simulink model "DYN_03x"  (R2021a)
(part 9 of 9)

C62 = 0.5*I6xx*de5*cos(e5)*sin(e4) - 0.5*I6xx*de4*cos(e4)*sin(e5) + 0.5*I6yy*de4*cos(e4)*sin(e5) - 0.5*I6yy*de5*cos(e5)*sin(e4) + I6zz*de4*cos(e4)*sin(e5) + I6zz*de5*cos(e5)*sin(e4) - 1.0*de2*m6*x6*y6*cos(e4)^2 + de2*m6*x6*y6*cos(e5)^2 - 1.0*de3*m6*x6*y6*cos(e4)^2 + de3*m6*x6*y6*cos(e5)^2 + 0.5*I6xx*de1*cos(e2)*cos(e3)*cos(e5) - 0.5*I6yy*de1*cos(e2)*cos(e3)*cos(e5) + I6xx*de2*cos(e4)*cos(e5)*sin(e4) + I6xx*de3*cos(e4)*cos(e5)*sin(e4) - 1.0*I6xx*de5*cos(e4)*cos(e6)*sin(e6) - 1.0*I6yy*de2*cos(e4)*cos(e5)*sin(e4) - 1.0*I6yy*de3*cos(e4)*cos(e5)*sin(e4) + I6yy*de5*cos(e4)*cos(e6)*sin(e6) - 0.5*I6xx*de1*cos(e5)*sin(e2)*sin(e3) + 0.5*I6yy*de1*cos(e5)*sin(e2)*sin(e3) + 1.5*de4*m6*x6^2*cos(e4)*sin(e5) + 0.5*de5*m6*x6^2*cos(e5)*sin(e4) + 0.5*de4*m6*y6^2*cos(e4)*sin(e5) + 1.5*de5*m6*y6^2*cos(e5)*sin(e4) - 1.0*I6xx*de2*cos(e4)^2*cos(e6)*sin(e6) + I6xx*de2*cos(e5)^2*cos(e6)*sin(e6) - 1.0*I6xx*de3*cos(e4)^2*cos(e6)*sin(e6) + I6xx*de4*cos(e4)*cos(e6)^2*sin(e5) + I6xx*de3*cos(e5)^2*cos(e6)*sin(e6) - 1.0*I6xx*de5*cos(e5)*cos(e6)^2*sin(e4) + I6yy*de2*cos(e4)^2*cos(e6)*sin(e6) - 1.0*I6yy*de2*cos(e5)^2*cos(e6)*sin(e6) + I6yy*de3*cos(e4)^2*cos(e6)*sin(e6) - 1.0*I6yy*de4*cos(e4)*cos(e6)^2*sin(e5) - 1.0*I6yy*de3*cos(e5)^2*cos(e6)*sin(e6) + I6yy*de5*cos(e5)*cos(e6)^2*sin(e4) - 1.0*de5*m6*x6*y6*cos(e4) + 2.0*de5*m6*x6*y6*cos(e4)*cos(e6)^2 + 0.5*I6xx*de1*cos(e2)*cos(e4)*sin(e3)*sin(e5) + 0.5*I6xx*de1*cos(e3)*cos(e4)*sin(e2)*sin(e5) - 0.5*I6yy*de1*cos(e2)*cos(e4)*sin(e3)*sin(e5) - 0.5*I6yy*de1*cos(e3)*cos(e4)*sin(e2)*sin(e5) - 0.5*de1*m6*x6^2*cos(e2)*cos(e3)*cos(e5) + 0.5*de1*m6*y6^2*cos(e2)*cos(e3)*cos(e5) - 1.0*de2*m6*x6^2*cos(e4)*cos(e5)*sin(e4) - 1.0*de3*m6*x6^2*cos(e4)*cos(e5)*sin(e4) + de5*m6*x6^2*cos(e4)*cos(e6)*sin(e6) - 1.0*de2*m6*x6*y6*cos(e4)^2*cos(e5)^2 + 2.0*de2*m6*x6*y6*cos(e4)^2*cos(e6)^2 - 1.0*de3*m6*x6*y6*cos(e4)^2*cos(e5)^2 - 2.0*de2*m6*x6*y6*cos(e5)^2*cos(e6)^2 + 2.0*de3*m6*x6*y6*cos(e4)^2*cos(e6)^2 - 2.0*de3*m6*x6*y6*cos(e5)^2*cos(e6)^2 + de2*m6*y6^2*cos(e4)*cos(e5)*sin(e4) + de3*m6*y6^2*cos(e4)*cos(e5)*sin(e4) - 1.0*de5*m6*y6^2*cos(e4)*cos(e6)*sin(e6) + 0.5*de1*m6*x6^2*cos(e5)*sin(e2)*sin(e3) - 0.5*de1*m6*y6^2*cos(e5)*sin(e2)*sin(e3) - 1.0*I6xx*de1*cos(e2)*cos(e3)*cos(e4)^2*cos(e5) - 1.0*I6xx*de1*cos(e2)*cos(e3)*cos(e5)*cos(e6)^2 + I6yy*de1*cos(e2)*cos(e3)*cos(e4)^2*cos(e5) + I6yy*de1*cos(e2)*cos(e3)*cos(e5)*cos(e6)^2 - 0.5*a3*de5*m6*y6*cos(e5)*cos(e6) + 0.5*d4*de4*m6*x6*cos(e4)*cos(e6) - 2.0*I6xx*de2*cos(e4)*cos(e5)*cos(e6)^2*sin(e4) - 2.0*I6xx*de3*cos(e4)*cos(e5)*cos(e6)^2*sin(e4) + 2.0*I6yy*de2*cos(e4)*cos(e5)*cos(e6)^2*sin(e4) + 2.0*I6yy*de3*cos(e4)*cos(e5)*cos(e6)^2*sin(e4) + a3*de2*m6*x6*cos(e6)*sin(e4) + a3*de3*m6*x6*cos(e6)*sin(e4) - 0.5*a3*de5*m6*x6*cos(e5)*sin(e6) - 0.5*a3*de6*m6*x6*cos(e6)*sin(e5) + I6xx*de1*cos(e4)^2*cos(e5)*sin(e2)*sin(e3) + I6xx*de1*cos(e5)*cos(e6)^2*sin(e2)*sin(e3) - 1.0*I6yy*de1*cos(e4)^2*cos(e5)*sin(e2)*sin(e3) - 1.0*I6yy*de1*cos(e5)*cos(e6)^2*sin(e2)*sin(e3) + d4*de2*m6*y6*cos(e6)*sin(e5) + d4*de3*m6*y6*cos(e6)*sin(e5) - 0.5*d4*de4*m6*y6*cos(e4)*sin(e6) - 0.5*d4*de6*m6*y6*cos(e6)*sin(e4) + 0.5*de6*m6*x6*z6*cos(e4)*cos(e6) - 1.0*a3*de2*m6*y6*sin(e4)*sin(e6) - 1.0*a3*de3*m6*y6*sin(e4)*sin(e6) + 0.5*a3*de6*m6*y6*sin(e5)*sin(e6) + d4*de2*m6*x6*sin(e5)*sin(e6) + d4*de3*m6*x6*sin(e5)*sin(e6) - 0.5*d4*de6*m6*x6*sin(e4)*sin(e6) - 1.5*de4*m6*y6*z6*cos(e6)*sin(e4) - 0.5*de6*m6*y6*z6*cos(e4)*sin(e6) + de2*m6*x6^2*cos(e4)^2*cos(e6)*sin(e6) - 1.0*de2*m6*x6^2*cos(e5)^2*cos(e6)*sin(e6) + de3*m6*x6^2*cos(e4)^2*cos(e6)*sin(e6) - 1.0*de4*m6*x6^2*cos(e4)*cos(e6)^2*sin(e5) - 1.0*de3*m6*x6^2*cos(e5)^2*cos(e6)*sin(e6) + de5*m6*x6^2*cos(e5)*cos(e6)^2*sin(e4) - 1.0*de2*m6*y6^2*cos(e4)^2*cos(e6)*sin(e6) + de2*m6*y6^2*cos(e5)^2*cos(e6)*sin(e6) - 1.0*de3*m6*y6^2*cos(e4)^2*cos(e6)*sin(e6) + de4*m6*y6^2*cos(e4)*cos(e6)^2*sin(e5) + de3*m6*y6^2*cos(e5)^2*cos(e6)*sin(e6) - 1.0*de5*m6*y6^2*cos(e5)*cos(e6)^2*sin(e4) - 1.5*de4*m6*x6*z6*sin(e4)*sin(e6) - 1.0*I6xx*de2*cos(e4)^2*cos(e5)^2*cos(e6)*sin(e6) - 1.0*I6xx*de3*cos(e4)^2*cos(e5)^2*cos(e6)*sin(e6) + I6yy*de2*cos(e4)^2*cos(e5)^2*cos(e6)*sin(e6) + I6yy*de3*cos(e4)^2*cos(e5)^2*cos(e6)*sin(e6) - 1.0*I6xx*de4*cos(e5)*cos(e6)*sin(e4)*sin(e5)*sin(e6) + I6yy*de4*cos(e5)*cos(e6)*sin(e4)*sin(e5)*sin(e6) - 0.5*de1*m6*x6^2*cos(e2)*cos(e4)*sin(e3)*sin(e5) - 0.5*de1*m6*x6^2*cos(e3)*cos(e4)*sin(e2)*sin(e5) + 0.5*de1*m6*y6^2*cos(e2)*cos(e4)*sin(e3)*sin(e5) + 0.5*de1*m6*y6^2*cos(e3)*cos(e4)*sin(e2)*sin(e5) - 0.5*a2*de1*m6*x6*cos(e2)*cos(e4)*cos(e6) + a3*de2*m6*y6*cos(e4)*cos(e5)*cos(e6) - 0.5*a2*de5*m6*y6*cos(e3)*cos(e5)*cos(e6) + a3*de3*m6*y6*cos(e4)*cos(e5)*cos(e6) + 0.5*d4*de6*m6*x6*cos(e4)*cos(e5)*cos(e6) + a2*de2*m6*x6*cos(e3)*cos(e6)*sin(e4) - 0.5*a2*de3*m6*x6*cos(e3)*cos(e6)*sin(e4) - 0.5*a2*de4*m6*x6*cos(e4)*cos(e6)*sin(e3) + a3*de2*m6*x6*cos(e4)*cos(e5)*sin(e6) - 0.5*a2*de5*m6*x6*cos(e3)*cos(e5)*sin(e6) + a3*de3*m6*x6*cos(e4)*cos(e5)*sin(e6) - 0.5*a2*de6*m6*x6*cos(e3)*cos(e6)*sin(e5) + 0.5*a2*de1*m6*y6*cos(e2)*cos(e4)*sin(e6) - 1.0*I6xx*de1*cos(e2)*cos(e4)*cos(e6)^2*sin(e3)*sin(e5) - 1.0*I6xx*de1*cos(e3)*cos(e4)*cos(e6)^2*sin(e2)*sin(e5) + I6yy*de1*cos(e2)*cos(e4)*cos(e6)^2*sin(e3)*sin(e5) + I6yy*de1*cos(e3)*cos(e4)*cos(e6)^2*sin(e2)*sin(e5) - 0.5*d4*de4*m6*y6*cos(e5)*cos(e6)*sin(e4) - 0.5*d4*de5*m6*y6*cos(e4)*cos(e6)*sin(e5) - 0.5*d4*de6*m6*y6*cos(e4)*cos(e5)*sin(e6) + 0.5*de4*m6*x6*z6*cos(e4)*cos(e5)*cos(e6) - 1.0*a2*de2*m6*y6*cos(e3)*sin(e4)*sin(e6) - 1.0*a2*de2*m6*y6*cos(e6)*sin(e3)*sin(e5) + 0.5*a2*de3*m6*y6*cos(e3)*sin(e4)*sin(e6) + 0.5*a2*de3*m6*y6*cos(e6)*sin(e3)*sin(e5) + 0.5*a2*de4*m6*y6*cos(e4)*sin(e3)*sin(e6) + 0.5*a2*de6*m6*y6*cos(e6)*sin(e3)*sin(e4) + 0.5*a2*de6*m6*y6*cos(e3)*sin(e5)*sin(e6) - 0.5*d4*de4*m6*x6*cos(e5)*sin(e4)*sin(e6) - 0.5*d4*de5*m6*x6*cos(e4)*sin(e5)*sin(e6) + de1*m6*x6^2*cos(e2)*cos(e3)*cos(e4)^2*cos(e5) + de1*m6*x6^2*cos(e2)*cos(e3)*cos(e5)*cos(e6)^2 - 1.0*de1*m6*y6^2*cos(e2)*cos(e3)*cos(e4)^2*cos(e5) - 1.0*de1*m6*y6^2*cos(e2)*cos(e3)*cos(e5)*cos(e6)^2 + de2*m6*y6*z6*cos(e5)*cos(e6)*sin(e5) + de3*m6*y6*z6*cos(e5)*cos(e6)*sin(e5) - 0.5*de4*m6*y6*z6*cos(e4)*cos(e5)*sin(e6) - 0.5*de6*m6*y6*z6*cos(e5)*cos(e6)*sin(e4) - 1.0*a2*de2*m6*x6*sin(e3)*sin(e5)*sin(e6) + 0.5*a2*de3*m6*x6*sin(e3)*sin(e5)*sin(e6) + 0.5*a2*de6*m6*x6*sin(e3)*sin(e4)*sin(e6) + 2.0*de2*m6*x6^2*cos(e4)*cos(e5)*cos(e6)^2*sin(e4) + 2.0*de3*m6*x6^2*cos(e4)*cos(e5)*cos(e6)^2*sin(e4) + 2.0*de2*m6*x6*y6*cos(e4)^2*cos(e5)^2*cos(e6)^2 + 2.0*de3*m6*x6*y6*cos(e4)^2*cos(e5)^2*cos(e6)^2 - 2.0*de2*m6*y6^2*cos(e4)*cos(e5)*cos(e6)^2*sin(e4) - 2.0*de3*m6*y6^2*cos(e4)*cos(e5)*cos(e6)^2*sin(e4) - 1.0*de4*m6*x6*y6*cos(e5)*sin(e4)*sin(e5) + de2*m6*x6*z6*cos(e5)*sin(e5)*sin(e6) + de3*m6*x6*z6*cos(e5)*sin(e5)*sin(e6) - 1.5*de5*m6*x6*z6*cos(e6)*sin(e4)*sin(e5) - 0.5*de6*m6*x6*z6*cos(e5)*sin(e4)*sin(e6) - 1.0*de1*m6*x6^2*cos(e4)^2*cos(e5)*sin(e2)*sin(e3) - 1.0*de1*m6*x6^2*cos(e5)*cos(e6)^2*sin(e2)*sin(e3) + de1*m6*y6^2*cos(e4)^2*cos(e5)*sin(e2)*sin(e3) + de1*m6*y6^2*cos(e5)*cos(e6)^2*sin(e2)*sin(e3) + 1.5*de5*m6*y6*z6*sin(e4)*sin(e5)*sin(e6) + 2.0*I6xx*de1*cos(e2)*cos(e3)*cos(e4)^2*cos(e5)*cos(e6)^2 - 2.0*I6yy*de1*cos(e2)*cos(e3)*cos(e4)^2*cos(e5)*cos(e6)^2 - 2.0*I6xx*de1*cos(e4)^2*cos(e5)*cos(e6)^2*sin(e2)*sin(e3) + 2.0*I6yy*de1*cos(e4)^2*cos(e5)*cos(e6)^2*sin(e2)*sin(e3) + de4*m6*y6*z6*cos(e5)^2*cos(e6)*sin(e4) + de2*m6*x6^2*cos(e4)^2*cos(e5)^2*cos(e6)*sin(e6) + de3*m6*x6^2*cos(e4)^2*cos(e5)^2*cos(e6)*sin(e6) - 1.0*de2*m6*y6^2*cos(e4)^2*cos(e5)^2*cos(e6)*sin(e6) - 1.0*de3*m6*y6^2*cos(e4)^2*cos(e5)^2*cos(e6)*sin(e6) + de4*m6*x6*z6*cos(e5)^2*sin(e4)*sin(e6) + de4*m6*x6^2*cos(e5)*cos(e6)*sin(e4)*sin(e5)*sin(e6) - 1.0*de4*m6*y6^2*cos(e5)*cos(e6)*sin(e4)*sin(e5)*sin(e6) - 0.5*a3*de1*m6*x6*cos(e2)*cos(e3)*cos(e4)*cos(e6) + a2*de2*m6*y6*cos(e3)*cos(e4)*cos(e5)*cos(e6) - 0.5*a2*de3*m6*y6*cos(e3)*cos(e4)*cos(e5)*cos(e6) + a2*de2*m6*x6*cos(e3)*cos(e4)*cos(e5)*sin(e6) - 0.5*a2*de3*m6*x6*cos(e3)*cos(e4)*cos(e5)*sin(e6) - 0.5*a2*de6*m6*x6*cos(e4)*cos(e5)*cos(e6)*sin(e3) + 0.5*a3*de1*m6*y6*cos(e2)*cos(e3)*cos(e4)*sin(e6) + 0.5*a2*de1*m6*y6*cos(e2)*cos(e5)*cos(e6)*sin(e4) + 0.5*d4*de1*m6*x6*cos(e2)*cos(e4)*cos(e6)*sin(e3) + 0.5*d4*de1*m6*x6*cos(e3)*cos(e4)*cos(e6)*sin(e2) + 0.5*a3*de1*m6*x6*cos(e4)*cos(e6)*sin(e2)*sin(e3) + 0.5*a2*de1*m6*x6*cos(e2)*cos(e5)*sin(e4)*sin(e6) + 0.5*a2*de4*m6*y6*cos(e5)*cos(e6)*sin(e3)*sin(e4) + 0.5*a2*de5*m6*y6*cos(e4)*cos(e6)*sin(e3)*sin(e5) + 0.5*a2*de6*m6*y6*cos(e4)*cos(e5)*sin(e3)*sin(e6) - 0.5*d4*de1*m6*y6*cos(e2)*cos(e4)*sin(e3)*sin(e6) - 0.5*d4*de1*m6*y6*cos(e3)*cos(e4)*sin(e2)*sin(e6) - 1.0*de1*m6*x6*y6*cos(e2)*cos(e3)*cos(e4)*sin(e4) - 0.5*de1*m6*x6*z6*cos(e2)*cos(e3)*cos(e6)*sin(e5) + 0.5*a2*de4*m6*x6*cos(e5)*sin(e3)*sin(e4)*sin(e6) + 0.5*a2*de5*m6*x6*cos(e4)*sin(e3)*sin(e5)*sin(e6) - 0.5*a3*de1*m6*y6*cos(e4)*sin(e2)*sin(e3)*sin(e6) + 2.0*de4*m6*x6*y6*cos(e4)*cos(e6)*sin(e5)*sin(e6) - 2.0*de5*m6*x6*y6*cos(e5)*cos(e6)*sin(e4)*sin(e6) - 1.0*de2*m6*x6*z6*cos(e4)*cos(e6)*sin(e4)*sin(e5) - 1.0*de3*m6*x6*z6*cos(e4)*cos(e6)*sin(e4)*sin(e5) + 0.5*de1*m6*y6*z6*cos(e2)*cos(e6)*sin(e3)*sin(e4) + 0.5*de1*m6*y6*z6*cos(e3)*cos(e6)*sin(e2)*sin(e4) + 0.5*de1*m6*y6*z6*cos(e2)*cos(e3)*sin(e5)*sin(e6) + de1*m6*x6^2*cos(e2)*cos(e4)*cos(e6)^2*sin(e3)*sin(e5) + de1*m6*x6^2*cos(e3)*cos(e4)*cos(e6)^2*sin(e2)*sin(e5) - 1.0*de1*m6*y6^2*cos(e2)*cos(e4)*cos(e6)^2*sin(e3)*sin(e5) - 1.0*de1*m6*y6^2*cos(e3)*cos(e4)*cos(e6)^2*sin(e2)*sin(e5) + de1*m6*x6*y6*cos(e4)*sin(e2)*sin(e3)*sin(e4) + 0.5*de1*m6*x6*z6*cos(e2)*sin(e3)*sin(e4)*sin(e6) + 0.5*de1*m6*x6*z6*cos(e3)*sin(e2)*sin(e4)*sin(e6) + 0.5*de1*m6*x6*z6*cos(e6)*sin(e2)*sin(e3)*sin(e5) + de2*m6*y6*z6*cos(e4)*sin(e4)*sin(e5)*sin(e6) + de3*m6*y6*z6*cos(e4)*sin(e4)*sin(e5)*sin(e6) - 0.5*de1*m6*y6*z6*sin(e2)*sin(e3)*sin(e5)*sin(e6) - 2.0*de1*m6*x6^2*cos(e2)*cos(e3)*cos(e4)^2*cos(e5)*cos(e6)^2 + 2.0*de1*m6*y6^2*cos(e2)*cos(e3)*cos(e4)^2*cos(e5)*cos(e6)^2 - 1.0*de2*m6*y6*z6*cos(e4)^2*cos(e5)*cos(e6)*sin(e5) - 1.0*de3*m6*y6*z6*cos(e4)^2*cos(e5)*cos(e6)*sin(e5) + 2.0*de4*m6*x6*y6*cos(e5)*cos(e6)^2*sin(e4)*sin(e5) - 1.0*de2*m6*x6*z6*cos(e4)^2*cos(e5)*sin(e5)*sin(e6) - 1.0*de3*m6*x6*z6*cos(e4)^2*cos(e5)*sin(e5)*sin(e6) + 2.0*de1*m6*x6^2*cos(e4)^2*cos(e5)*cos(e6)^2*sin(e2)*sin(e3) - 2.0*de1*m6*y6^2*cos(e4)^2*cos(e5)*cos(e6)^2*sin(e2)*sin(e3) - 1.0*I6xx*de1*cos(e2)*cos(e3)*cos(e4)*cos(e6)*sin(e4)*sin(e6) + I6yy*de1*cos(e2)*cos(e3)*cos(e4)*cos(e6)*sin(e4)*sin(e6) + I6xx*de1*cos(e4)*cos(e6)*sin(e2)*sin(e3)*sin(e4)*sin(e6) - 1.0*I6yy*de1*cos(e4)*cos(e6)*sin(e2)*sin(e3)*sin(e4)*sin(e6) + 0.5*a3*de1*m6*y6*cos(e2)*cos(e3)*cos(e5)*cos(e6)*sin(e4) - 1.0*I6xx*de1*cos(e2)*cos(e3)*cos(e4)*cos(e5)^2*cos(e6)*sin(e4)*sin(e6) + I6yy*de1*cos(e2)*cos(e3)*cos(e4)*cos(e5)^2*cos(e6)*sin(e4)*sin(e6) + 0.5*a3*de1*m6*x6*cos(e2)*cos(e3)*cos(e5)*sin(e4)*sin(e6) - 0.5*d4*de1*m6*y6*cos(e2)*cos(e5)*cos(e6)*sin(e3)*sin(e4) - 0.5*d4*de1*m6*y6*cos(e3)*cos(e5)*cos(e6)*sin(e2)*sin(e4) - 2.0*de1*m6*x6*y6*cos(e2)*cos(e3)*cos(e5)*cos(e6)*sin(e6) + 0.5*de1*m6*x6*z6*cos(e2)*cos(e4)*cos(e5)*cos(e6)*sin(e3) + 0.5*de1*m6*x6*z6*cos(e3)*cos(e4)*cos(e5)*cos(e6)*sin(e2) - 0.5*a3*de1*m6*y6*cos(e5)*cos(e6)*sin(e2)*sin(e3)*sin(e4) - 0.5*d4*de1*m6*x6*cos(e2)*cos(e5)*sin(e3)*sin(e4)*sin(e6) - 0.5*d4*de1*m6*x6*cos(e3)*cos(e5)*sin(e2)*sin(e4)*sin(e6) + I6xx*de1*cos(e4)*cos(e5)^2*cos(e6)*sin(e2)*sin(e3)*sin(e4)*sin(e6) - 1.0*I6yy*de1*cos(e4)*cos(e5)^2*cos(e6)*sin(e2)*sin(e3)*sin(e4)*sin(e6) - 4.0*de2*m6*x6*y6*cos(e4)*cos(e5)*cos(e6)*sin(e4)*sin(e6) - 4.0*de3*m6*x6*y6*cos(e4)*cos(e5)*cos(e6)*sin(e4)*sin(e6) - 0.5*de1*m6*y6*z6*cos(e2)*cos(e4)*cos(e5)*sin(e3)*sin(e6) - 0.5*de1*m6*y6*z6*cos(e3)*cos(e4)*cos(e5)*sin(e2)*sin(e6) - 0.5*a3*de1*m6*x6*cos(e5)*sin(e2)*sin(e3)*sin(e4)*sin(e6) + de1*m6*x6*y6*cos(e2)*cos(e5)*sin(e3)*sin(e4)*sin(e5) + de1*m6*x6*y6*cos(e3)*cos(e5)*sin(e2)*sin(e4)*sin(e5) + 2.0*de1*m6*x6*y6*cos(e5)*cos(e6)*sin(e2)*sin(e3)*sin(e6) - 1.0*de1*m6*x6*y6*cos(e2)*cos(e3)*cos(e4)*cos(e5)^2*sin(e4) + 2.0*de1*m6*x6*y6*cos(e2)*cos(e3)*cos(e4)*cos(e6)^2*sin(e4) + de1*m6*x6*z6*cos(e2)*cos(e3)*cos(e4)^2*cos(e6)*sin(e5) - 1.0*de1*m6*y6*z6*cos(e2)*cos(e3)*cos(e4)^2*sin(e5)*sin(e6) - 1.0*de1*m6*y6*z6*cos(e2)*cos(e5)^2*cos(e6)*sin(e3)*sin(e4) - 1.0*de1*m6*y6*z6*cos(e3)*cos(e5)^2*cos(e6)*sin(e2)*sin(e4) + de1*m6*x6*y6*cos(e4)*cos(e5)^2*sin(e2)*sin(e3)*sin(e4) - 2.0*de1*m6*x6*y6*cos(e4)*cos(e6)^2*sin(e2)*sin(e3)*sin(e4) - 1.0*de1*m6*x6*z6*cos(e2)*cos(e5)^2*sin(e3)*sin(e4)*sin(e6) - 1.0*de1*m6*x6*z6*cos(e3)*cos(e5)^2*sin(e2)*sin(e4)*sin(e6) - 1.0*de1*m6*x6*z6*cos(e4)^2*cos(e6)*sin(e2)*sin(e3)*sin(e5) + de1*m6*y6*z6*cos(e4)^2*sin(e2)*sin(e3)*sin(e5)*sin(e6) + I6xx*de1*cos(e2)*cos(e5)*cos(e6)*sin(e3)*sin(e4)*sin(e5)*sin(e6) + I6xx*de1*cos(e3)*cos(e5)*cos(e6)*sin(e2)*sin(e4)*sin(e5)*sin(e6) - 1.0*I6yy*de1*cos(e2)*cos(e5)*cos(e6)*sin(e3)*sin(e4)*sin(e5)*sin(e6) - 1.0*I6yy*de1*cos(e3)*cos(e5)*cos(e6)*sin(e2)*sin(e4)*sin(e5)*sin(e6) + de1*m6*x6^2*cos(e2)*cos(e3)*cos(e4)*cos(e6)*sin(e4)*sin(e6) - 1.0*de1*m6*y6^2*cos(e2)*cos(e3)*cos(e4)*cos(e6)*sin(e4)*sin(e6) - 1.0*de1*m6*x6^2*cos(e4)*cos(e6)*sin(e2)*sin(e3)*sin(e4)*sin(e6) + de1*m6*y6^2*cos(e4)*cos(e6)*sin(e2)*sin(e3)*sin(e4)*sin(e6) + de1*m6*x6^2*cos(e2)*cos(e3)*cos(e4)*cos(e5)^2*cos(e6)*sin(e4)*sin(e6) - 1.0*de1*m6*y6^2*cos(e2)*cos(e3)*cos(e4)*cos(e5)^2*cos(e6)*sin(e4)*sin(e6) - 2.0*de1*m6*x6*y6*cos(e2)*cos(e4)*cos(e6)*sin(e3)*sin(e5)*sin(e6) - 2.0*de1*m6*x6*y6*cos(e3)*cos(e4)*cos(e6)*sin(e2)*sin(e5)*sin(e6) - 1.0*de1*m6*x6^2*cos(e4)*cos(e5)^2*cos(e6)*sin(e2)*sin(e3)*sin(e4)*sin(e6) + de1*m6*y6^2*cos(e4)*cos(e5)^2*cos(e6)*sin(e2)*sin(e3)*sin(e4)*sin(e6) + 4.0*de1*m6*x6*y6*cos(e2)*cos(e3)*cos(e4)^2*cos(e5)*cos(e6)*sin(e6) - 2.0*de1*m6*x6*y6*cos(e2)*cos(e5)*cos(e6)^2*sin(e3)*sin(e4)*sin(e5) - 2.0*de1*m6*x6*y6*cos(e3)*cos(e5)*cos(e6)^2*sin(e2)*sin(e4)*sin(e5) - 4.0*de1*m6*x6*y6*cos(e4)^2*cos(e5)*cos(e6)*sin(e2)*sin(e3)*sin(e6) + 2.0*de1*m6*x6*y6*cos(e2)*cos(e3)*cos(e4)*cos(e5)^2*cos(e6)^2*sin(e4) - 1.0*de1*m6*x6^2*cos(e2)*cos(e5)*cos(e6)*sin(e3)*sin(e4)*sin(e5)*sin(e6) - 1.0*de1*m6*x6^2*cos(e3)*cos(e5)*cos(e6)*sin(e2)*sin(e4)*sin(e5)*sin(e6) - 2.0*de1*m6*x6*y6*cos(e4)*cos(e5)^2*cos(e6)^2*sin(e2)*sin(e3)*sin(e4) + de1*m6*y6^2*cos(e2)*cos(e5)*cos(e6)*sin(e3)*sin(e4)*sin(e5)*sin(e6) + de1*m6*y6^2*cos(e3)*cos(e5)*cos(e6)*sin(e2)*sin(e4)*sin(e5)*sin(e6) - 1.0*de1*m6*y6*z6*cos(e2)*cos(e3)*cos(e4)*cos(e5)*cos(e6)*sin(e4)*sin(e5) - 1.0*de1*m6*x6*z6*cos(e2)*cos(e3)*cos(e4)*cos(e5)*sin(e4)*sin(e5)*sin(e6) + de1*m6*y6*z6*cos(e4)*cos(e5)*cos(e6)*sin(e2)*sin(e3)*sin(e4)*sin(e5) + de1*m6*x6*z6*cos(e4)*cos(e5)*sin(e2)*sin(e3)*sin(e4)*sin(e5)*sin(e6);
C63 = 0.5*I6xx*de5*cos(e5)*sin(e4) - 0.5*I6xx*de4*cos(e4)*sin(e5) + 0.5*I6yy*de4*cos(e4)*sin(e5) - 0.5*I6yy*de5*cos(e5)*sin(e4) + I6zz*de4*cos(e4)*sin(e5) + I6zz*de5*cos(e5)*sin(e4) - 1.0*de2*m6*x6*y6*cos(e4)^2 + de2*m6*x6*y6*cos(e5)^2 - 1.0*de3*m6*x6*y6*cos(e4)^2 + de3*m6*x6*y6*cos(e5)^2 + 0.5*I6xx*de1*cos(e2)*cos(e3)*cos(e5) - 0.5*I6yy*de1*cos(e2)*cos(e3)*cos(e5) + I6xx*de2*cos(e4)*cos(e5)*sin(e4) + I6xx*de3*cos(e4)*cos(e5)*sin(e4) - 1.0*I6xx*de5*cos(e4)*cos(e6)*sin(e6) - 1.0*I6yy*de2*cos(e4)*cos(e5)*sin(e4) - 1.0*I6yy*de3*cos(e4)*cos(e5)*sin(e4) + I6yy*de5*cos(e4)*cos(e6)*sin(e6) - 0.5*I6xx*de1*cos(e5)*sin(e2)*sin(e3) + 0.5*I6yy*de1*cos(e5)*sin(e2)*sin(e3) + 1.5*de4*m6*x6^2*cos(e4)*sin(e5) + 0.5*de5*m6*x6^2*cos(e5)*sin(e4) + 0.5*de4*m6*y6^2*cos(e4)*sin(e5) + 1.5*de5*m6*y6^2*cos(e5)*sin(e4) - 1.0*I6xx*de2*cos(e4)^2*cos(e6)*sin(e6) + I6xx*de2*cos(e5)^2*cos(e6)*sin(e6) - 1.0*I6xx*de3*cos(e4)^2*cos(e6)*sin(e6) + I6xx*de4*cos(e4)*cos(e6)^2*sin(e5) + I6xx*de3*cos(e5)^2*cos(e6)*sin(e6) - 1.0*I6xx*de5*cos(e5)*cos(e6)^2*sin(e4) + I6yy*de2*cos(e4)^2*cos(e6)*sin(e6) - 1.0*I6yy*de2*cos(e5)^2*cos(e6)*sin(e6) + I6yy*de3*cos(e4)^2*cos(e6)*sin(e6) - 1.0*I6yy*de4*cos(e4)*cos(e6)^2*sin(e5) - 1.0*I6yy*de3*cos(e5)^2*cos(e6)*sin(e6) + I6yy*de5*cos(e5)*cos(e6)^2*sin(e4) - 1.0*de5*m6*x6*y6*cos(e4) + 2.0*de5*m6*x6*y6*cos(e4)*cos(e6)^2 + 0.5*I6xx*de1*cos(e2)*cos(e4)*sin(e3)*sin(e5) + 0.5*I6xx*de1*cos(e3)*cos(e4)*sin(e2)*sin(e5) - 0.5*I6yy*de1*cos(e2)*cos(e4)*sin(e3)*sin(e5) - 0.5*I6yy*de1*cos(e3)*cos(e4)*sin(e2)*sin(e5) - 0.5*de1*m6*x6^2*cos(e2)*cos(e3)*cos(e5) + 0.5*de1*m6*y6^2*cos(e2)*cos(e3)*cos(e5) - 1.0*de2*m6*x6^2*cos(e4)*cos(e5)*sin(e4) - 1.0*de3*m6*x6^2*cos(e4)*cos(e5)*sin(e4) + de5*m6*x6^2*cos(e4)*cos(e6)*sin(e6) - 1.0*de2*m6*x6*y6*cos(e4)^2*cos(e5)^2 + 2.0*de2*m6*x6*y6*cos(e4)^2*cos(e6)^2 - 1.0*de3*m6*x6*y6*cos(e4)^2*cos(e5)^2 - 2.0*de2*m6*x6*y6*cos(e5)^2*cos(e6)^2 + 2.0*de3*m6*x6*y6*cos(e4)^2*cos(e6)^2 - 2.0*de3*m6*x6*y6*cos(e5)^2*cos(e6)^2 + de2*m6*y6^2*cos(e4)*cos(e5)*sin(e4) + de3*m6*y6^2*cos(e4)*cos(e5)*sin(e4) - 1.0*de5*m6*y6^2*cos(e4)*cos(e6)*sin(e6) + 0.5*de1*m6*x6^2*cos(e5)*sin(e2)*sin(e3) - 0.5*de1*m6*y6^2*cos(e5)*sin(e2)*sin(e3) - 1.0*I6xx*de1*cos(e2)*cos(e3)*cos(e4)^2*cos(e5) - 1.0*I6xx*de1*cos(e2)*cos(e3)*cos(e5)*cos(e6)^2 + I6yy*de1*cos(e2)*cos(e3)*cos(e4)^2*cos(e5) + I6yy*de1*cos(e2)*cos(e3)*cos(e5)*cos(e6)^2 - 0.5*a3*de5*m6*y6*cos(e5)*cos(e6) + 0.5*d4*de4*m6*x6*cos(e4)*cos(e6) - 2.0*I6xx*de2*cos(e4)*cos(e5)*cos(e6)^2*sin(e4) - 2.0*I6xx*de3*cos(e4)*cos(e5)*cos(e6)^2*sin(e4) + 2.0*I6yy*de2*cos(e4)*cos(e5)*cos(e6)^2*sin(e4) + 2.0*I6yy*de3*cos(e4)*cos(e5)*cos(e6)^2*sin(e4) + a3*de2*m6*x6*cos(e6)*sin(e4) + a3*de3*m6*x6*cos(e6)*sin(e4) - 0.5*a3*de5*m6*x6*cos(e5)*sin(e6) - 0.5*a3*de6*m6*x6*cos(e6)*sin(e5) + I6xx*de1*cos(e4)^2*cos(e5)*sin(e2)*sin(e3) + I6xx*de1*cos(e5)*cos(e6)^2*sin(e2)*sin(e3) - 1.0*I6yy*de1*cos(e4)^2*cos(e5)*sin(e2)*sin(e3) - 1.0*I6yy*de1*cos(e5)*cos(e6)^2*sin(e2)*sin(e3) + d4*de2*m6*y6*cos(e6)*sin(e5) + d4*de3*m6*y6*cos(e6)*sin(e5) - 0.5*d4*de4*m6*y6*cos(e4)*sin(e6) - 0.5*d4*de6*m6*y6*cos(e6)*sin(e4) + 0.5*de6*m6*x6*z6*cos(e4)*cos(e6) - 1.0*a3*de2*m6*y6*sin(e4)*sin(e6) - 1.0*a3*de3*m6*y6*sin(e4)*sin(e6) + 0.5*a3*de6*m6*y6*sin(e5)*sin(e6) + d4*de2*m6*x6*sin(e5)*sin(e6) + d4*de3*m6*x6*sin(e5)*sin(e6) - 0.5*d4*de6*m6*x6*sin(e4)*sin(e6) - 1.5*de4*m6*y6*z6*cos(e6)*sin(e4) - 0.5*de6*m6*y6*z6*cos(e4)*sin(e6) + de2*m6*x6^2*cos(e4)^2*cos(e6)*sin(e6) - 1.0*de2*m6*x6^2*cos(e5)^2*cos(e6)*sin(e6) + de3*m6*x6^2*cos(e4)^2*cos(e6)*sin(e6) - 1.0*de4*m6*x6^2*cos(e4)*cos(e6)^2*sin(e5) - 1.0*de3*m6*x6^2*cos(e5)^2*cos(e6)*sin(e6) + de5*m6*x6^2*cos(e5)*cos(e6)^2*sin(e4) - 1.0*de2*m6*y6^2*cos(e4)^2*cos(e6)*sin(e6) + de2*m6*y6^2*cos(e5)^2*cos(e6)*sin(e6) - 1.0*de3*m6*y6^2*cos(e4)^2*cos(e6)*sin(e6) + de4*m6*y6^2*cos(e4)*cos(e6)^2*sin(e5) + de3*m6*y6^2*cos(e5)^2*cos(e6)*sin(e6) - 1.0*de5*m6*y6^2*cos(e5)*cos(e6)^2*sin(e4) - 1.5*de4*m6*x6*z6*sin(e4)*sin(e6) - 1.0*I6xx*de2*cos(e4)^2*cos(e5)^2*cos(e6)*sin(e6) - 1.0*I6xx*de3*cos(e4)^2*cos(e5)^2*cos(e6)*sin(e6) + I6yy*de2*cos(e4)^2*cos(e5)^2*cos(e6)*sin(e6) + I6yy*de3*cos(e4)^2*cos(e5)^2*cos(e6)*sin(e6) - 1.0*I6xx*de4*cos(e5)*cos(e6)*sin(e4)*sin(e5)*sin(e6) + I6yy*de4*cos(e5)*cos(e6)*sin(e4)*sin(e5)*sin(e6) - 0.5*de1*m6*x6^2*cos(e2)*cos(e4)*sin(e3)*sin(e5) - 0.5*de1*m6*x6^2*cos(e3)*cos(e4)*sin(e2)*sin(e5) + 0.5*de1*m6*y6^2*cos(e2)*cos(e4)*sin(e3)*sin(e5) + 0.5*de1*m6*y6^2*cos(e3)*cos(e4)*sin(e2)*sin(e5) + a3*de2*m6*y6*cos(e4)*cos(e5)*cos(e6) + a3*de3*m6*y6*cos(e4)*cos(e5)*cos(e6) + 0.5*d4*de6*m6*x6*cos(e4)*cos(e5)*cos(e6) + 0.5*a2*de2*m6*x6*cos(e3)*cos(e6)*sin(e4) + a3*de2*m6*x6*cos(e4)*cos(e5)*sin(e6) + a3*de3*m6*x6*cos(e4)*cos(e5)*sin(e6) - 1.0*I6xx*de1*cos(e2)*cos(e4)*cos(e6)^2*sin(e3)*sin(e5) - 1.0*I6xx*de1*cos(e3)*cos(e4)*cos(e6)^2*sin(e2)*sin(e5) + I6yy*de1*cos(e2)*cos(e4)*cos(e6)^2*sin(e3)*sin(e5) + I6yy*de1*cos(e3)*cos(e4)*cos(e6)^2*sin(e2)*sin(e5) - 0.5*d4*de4*m6*y6*cos(e5)*cos(e6)*sin(e4) - 0.5*d4*de5*m6*y6*cos(e4)*cos(e6)*sin(e5) - 0.5*d4*de6*m6*y6*cos(e4)*cos(e5)*sin(e6) + 0.5*de4*m6*x6*z6*cos(e4)*cos(e5)*cos(e6) - 0.5*a2*de2*m6*y6*cos(e3)*sin(e4)*sin(e6) - 0.5*a2*de2*m6*y6*cos(e6)*sin(e3)*sin(e5) - 0.5*d4*de4*m6*x6*cos(e5)*sin(e4)*sin(e6) - 0.5*d4*de5*m6*x6*cos(e4)*sin(e5)*sin(e6) + de1*m6*x6^2*cos(e2)*cos(e3)*cos(e4)^2*cos(e5) + de1*m6*x6^2*cos(e2)*cos(e3)*cos(e5)*cos(e6)^2 - 1.0*de1*m6*y6^2*cos(e2)*cos(e3)*cos(e4)^2*cos(e5) - 1.0*de1*m6*y6^2*cos(e2)*cos(e3)*cos(e5)*cos(e6)^2 + de2*m6*y6*z6*cos(e5)*cos(e6)*sin(e5) + de3*m6*y6*z6*cos(e5)*cos(e6)*sin(e5) - 0.5*de4*m6*y6*z6*cos(e4)*cos(e5)*sin(e6) - 0.5*de6*m6*y6*z6*cos(e5)*cos(e6)*sin(e4) - 0.5*a2*de2*m6*x6*sin(e3)*sin(e5)*sin(e6) + 2.0*de2*m6*x6^2*cos(e4)*cos(e5)*cos(e6)^2*sin(e4) + 2.0*de3*m6*x6^2*cos(e4)*cos(e5)*cos(e6)^2*sin(e4) + 2.0*de2*m6*x6*y6*cos(e4)^2*cos(e5)^2*cos(e6)^2 + 2.0*de3*m6*x6*y6*cos(e4)^2*cos(e5)^2*cos(e6)^2 - 2.0*de2*m6*y6^2*cos(e4)*cos(e5)*cos(e6)^2*sin(e4) - 2.0*de3*m6*y6^2*cos(e4)*cos(e5)*cos(e6)^2*sin(e4) - 1.0*de4*m6*x6*y6*cos(e5)*sin(e4)*sin(e5) + de2*m6*x6*z6*cos(e5)*sin(e5)*sin(e6) + de3*m6*x6*z6*cos(e5)*sin(e5)*sin(e6) - 1.5*de5*m6*x6*z6*cos(e6)*sin(e4)*sin(e5) - 0.5*de6*m6*x6*z6*cos(e5)*sin(e4)*sin(e6) - 1.0*de1*m6*x6^2*cos(e4)^2*cos(e5)*sin(e2)*sin(e3) - 1.0*de1*m6*x6^2*cos(e5)*cos(e6)^2*sin(e2)*sin(e3) + de1*m6*y6^2*cos(e4)^2*cos(e5)*sin(e2)*sin(e3) + de1*m6*y6^2*cos(e5)*cos(e6)^2*sin(e2)*sin(e3) + 1.5*de5*m6*y6*z6*sin(e4)*sin(e5)*sin(e6) + 2.0*I6xx*de1*cos(e2)*cos(e3)*cos(e4)^2*cos(e5)*cos(e6)^2 - 2.0*I6yy*de1*cos(e2)*cos(e3)*cos(e4)^2*cos(e5)*cos(e6)^2 - 2.0*I6xx*de1*cos(e4)^2*cos(e5)*cos(e6)^2*sin(e2)*sin(e3) + 2.0*I6yy*de1*cos(e4)^2*cos(e5)*cos(e6)^2*sin(e2)*sin(e3) + de4*m6*y6*z6*cos(e5)^2*cos(e6)*sin(e4) + de2*m6*x6^2*cos(e4)^2*cos(e5)^2*cos(e6)*sin(e6) + de3*m6*x6^2*cos(e4)^2*cos(e5)^2*cos(e6)*sin(e6) - 1.0*de2*m6*y6^2*cos(e4)^2*cos(e5)^2*cos(e6)*sin(e6) - 1.0*de3*m6*y6^2*cos(e4)^2*cos(e5)^2*cos(e6)*sin(e6) + de4*m6*x6*z6*cos(e5)^2*sin(e4)*sin(e6) + de4*m6*x6^2*cos(e5)*cos(e6)*sin(e4)*sin(e5)*sin(e6) - 1.0*de4*m6*y6^2*cos(e5)*cos(e6)*sin(e4)*sin(e5)*sin(e6) - 0.5*a3*de1*m6*x6*cos(e2)*cos(e3)*cos(e4)*cos(e6) + 0.5*a2*de2*m6*y6*cos(e3)*cos(e4)*cos(e5)*cos(e6) + 0.5*a2*de2*m6*x6*cos(e3)*cos(e4)*cos(e5)*sin(e6) + 0.5*a3*de1*m6*y6*cos(e2)*cos(e3)*cos(e4)*sin(e6) + 0.5*d4*de1*m6*x6*cos(e2)*cos(e4)*cos(e6)*sin(e3) + 0.5*d4*de1*m6*x6*cos(e3)*cos(e4)*cos(e6)*sin(e2) + 0.5*a3*de1*m6*x6*cos(e4)*cos(e6)*sin(e2)*sin(e3) - 0.5*d4*de1*m6*y6*cos(e2)*cos(e4)*sin(e3)*sin(e6) - 0.5*d4*de1*m6*y6*cos(e3)*cos(e4)*sin(e2)*sin(e6) - 1.0*de1*m6*x6*y6*cos(e2)*cos(e3)*cos(e4)*sin(e4) - 0.5*de1*m6*x6*z6*cos(e2)*cos(e3)*cos(e6)*sin(e5) - 0.5*a3*de1*m6*y6*cos(e4)*sin(e2)*sin(e3)*sin(e6) + 2.0*de4*m6*x6*y6*cos(e4)*cos(e6)*sin(e5)*sin(e6) - 2.0*de5*m6*x6*y6*cos(e5)*cos(e6)*sin(e4)*sin(e6) - 1.0*de2*m6*x6*z6*cos(e4)*cos(e6)*sin(e4)*sin(e5) - 1.0*de3*m6*x6*z6*cos(e4)*cos(e6)*sin(e4)*sin(e5) + 0.5*de1*m6*y6*z6*cos(e2)*cos(e6)*sin(e3)*sin(e4) + 0.5*de1*m6*y6*z6*cos(e3)*cos(e6)*sin(e2)*sin(e4) + 0.5*de1*m6*y6*z6*cos(e2)*cos(e3)*sin(e5)*sin(e6) + de1*m6*x6^2*cos(e2)*cos(e4)*cos(e6)^2*sin(e3)*sin(e5) + de1*m6*x6^2*cos(e3)*cos(e4)*cos(e6)^2*sin(e2)*sin(e5) - 1.0*de1*m6*y6^2*cos(e2)*cos(e4)*cos(e6)^2*sin(e3)*sin(e5) - 1.0*de1*m6*y6^2*cos(e3)*cos(e4)*cos(e6)^2*sin(e2)*sin(e5) + de1*m6*x6*y6*cos(e4)*sin(e2)*sin(e3)*sin(e4) + 0.5*de1*m6*x6*z6*cos(e2)*sin(e3)*sin(e4)*sin(e6) + 0.5*de1*m6*x6*z6*cos(e3)*sin(e2)*sin(e4)*sin(e6) + 0.5*de1*m6*x6*z6*cos(e6)*sin(e2)*sin(e3)*sin(e5) + de2*m6*y6*z6*cos(e4)*sin(e4)*sin(e5)*sin(e6) + de3*m6*y6*z6*cos(e4)*sin(e4)*sin(e5)*sin(e6) - 0.5*de1*m6*y6*z6*sin(e2)*sin(e3)*sin(e5)*sin(e6) - 2.0*de1*m6*x6^2*cos(e2)*cos(e3)*cos(e4)^2*cos(e5)*cos(e6)^2 + 2.0*de1*m6*y6^2*cos(e2)*cos(e3)*cos(e4)^2*cos(e5)*cos(e6)^2 - 1.0*de2*m6*y6*z6*cos(e4)^2*cos(e5)*cos(e6)*sin(e5) - 1.0*de3*m6*y6*z6*cos(e4)^2*cos(e5)*cos(e6)*sin(e5) + 2.0*de4*m6*x6*y6*cos(e5)*cos(e6)^2*sin(e4)*sin(e5) - 1.0*de2*m6*x6*z6*cos(e4)^2*cos(e5)*sin(e5)*sin(e6) - 1.0*de3*m6*x6*z6*cos(e4)^2*cos(e5)*sin(e5)*sin(e6) + 2.0*de1*m6*x6^2*cos(e4)^2*cos(e5)*cos(e6)^2*sin(e2)*sin(e3) - 2.0*de1*m6*y6^2*cos(e4)^2*cos(e5)*cos(e6)^2*sin(e2)*sin(e3) - 1.0*I6xx*de1*cos(e2)*cos(e3)*cos(e4)*cos(e6)*sin(e4)*sin(e6) + I6yy*de1*cos(e2)*cos(e3)*cos(e4)*cos(e6)*sin(e4)*sin(e6) + I6xx*de1*cos(e4)*cos(e6)*sin(e2)*sin(e3)*sin(e4)*sin(e6) - 1.0*I6yy*de1*cos(e4)*cos(e6)*sin(e2)*sin(e3)*sin(e4)*sin(e6) + 0.5*a3*de1*m6*y6*cos(e2)*cos(e3)*cos(e5)*cos(e6)*sin(e4) - 1.0*I6xx*de1*cos(e2)*cos(e3)*cos(e4)*cos(e5)^2*cos(e6)*sin(e4)*sin(e6) + I6yy*de1*cos(e2)*cos(e3)*cos(e4)*cos(e5)^2*cos(e6)*sin(e4)*sin(e6) + 0.5*a3*de1*m6*x6*cos(e2)*cos(e3)*cos(e5)*sin(e4)*sin(e6) - 0.5*d4*de1*m6*y6*cos(e2)*cos(e5)*cos(e6)*sin(e3)*sin(e4) - 0.5*d4*de1*m6*y6*cos(e3)*cos(e5)*cos(e6)*sin(e2)*sin(e4) - 2.0*de1*m6*x6*y6*cos(e2)*cos(e3)*cos(e5)*cos(e6)*sin(e6) + 0.5*de1*m6*x6*z6*cos(e2)*cos(e4)*cos(e5)*cos(e6)*sin(e3) + 0.5*de1*m6*x6*z6*cos(e3)*cos(e4)*cos(e5)*cos(e6)*sin(e2) - 0.5*a3*de1*m6*y6*cos(e5)*cos(e6)*sin(e2)*sin(e3)*sin(e4) - 0.5*d4*de1*m6*x6*cos(e2)*cos(e5)*sin(e3)*sin(e4)*sin(e6) - 0.5*d4*de1*m6*x6*cos(e3)*cos(e5)*sin(e2)*sin(e4)*sin(e6) + I6xx*de1*cos(e4)*cos(e5)^2*cos(e6)*sin(e2)*sin(e3)*sin(e4)*sin(e6) - 1.0*I6yy*de1*cos(e4)*cos(e5)^2*cos(e6)*sin(e2)*sin(e3)*sin(e4)*sin(e6) - 4.0*de2*m6*x6*y6*cos(e4)*cos(e5)*cos(e6)*sin(e4)*sin(e6) - 4.0*de3*m6*x6*y6*cos(e4)*cos(e5)*cos(e6)*sin(e4)*sin(e6) - 0.5*de1*m6*y6*z6*cos(e2)*cos(e4)*cos(e5)*sin(e3)*sin(e6) - 0.5*de1*m6*y6*z6*cos(e3)*cos(e4)*cos(e5)*sin(e2)*sin(e6) - 0.5*a3*de1*m6*x6*cos(e5)*sin(e2)*sin(e3)*sin(e4)*sin(e6) + de1*m6*x6*y6*cos(e2)*cos(e5)*sin(e3)*sin(e4)*sin(e5) + de1*m6*x6*y6*cos(e3)*cos(e5)*sin(e2)*sin(e4)*sin(e5) + 2.0*de1*m6*x6*y6*cos(e5)*cos(e6)*sin(e2)*sin(e3)*sin(e6) - 1.0*de1*m6*x6*y6*cos(e2)*cos(e3)*cos(e4)*cos(e5)^2*sin(e4) + 2.0*de1*m6*x6*y6*cos(e2)*cos(e3)*cos(e4)*cos(e6)^2*sin(e4) + de1*m6*x6*z6*cos(e2)*cos(e3)*cos(e4)^2*cos(e6)*sin(e5) - 1.0*de1*m6*y6*z6*cos(e2)*cos(e3)*cos(e4)^2*sin(e5)*sin(e6) - 1.0*de1*m6*y6*z6*cos(e2)*cos(e5)^2*cos(e6)*sin(e3)*sin(e4) - 1.0*de1*m6*y6*z6*cos(e3)*cos(e5)^2*cos(e6)*sin(e2)*sin(e4) + de1*m6*x6*y6*cos(e4)*cos(e5)^2*sin(e2)*sin(e3)*sin(e4) - 2.0*de1*m6*x6*y6*cos(e4)*cos(e6)^2*sin(e2)*sin(e3)*sin(e4) - 1.0*de1*m6*x6*z6*cos(e2)*cos(e5)^2*sin(e3)*sin(e4)*sin(e6) - 1.0*de1*m6*x6*z6*cos(e3)*cos(e5)^2*sin(e2)*sin(e4)*sin(e6) - 1.0*de1*m6*x6*z6*cos(e4)^2*cos(e6)*sin(e2)*sin(e3)*sin(e5) + de1*m6*y6*z6*cos(e4)^2*sin(e2)*sin(e3)*sin(e5)*sin(e6) + I6xx*de1*cos(e2)*cos(e5)*cos(e6)*sin(e3)*sin(e4)*sin(e5)*sin(e6) + I6xx*de1*cos(e3)*cos(e5)*cos(e6)*sin(e2)*sin(e4)*sin(e5)*sin(e6) - 1.0*I6yy*de1*cos(e2)*cos(e5)*cos(e6)*sin(e3)*sin(e4)*sin(e5)*sin(e6) - 1.0*I6yy*de1*cos(e3)*cos(e5)*cos(e6)*sin(e2)*sin(e4)*sin(e5)*sin(e6) + de1*m6*x6^2*cos(e2)*cos(e3)*cos(e4)*cos(e6)*sin(e4)*sin(e6) - 1.0*de1*m6*y6^2*cos(e2)*cos(e3)*cos(e4)*cos(e6)*sin(e4)*sin(e6) - 1.0*de1*m6*x6^2*cos(e4)*cos(e6)*sin(e2)*sin(e3)*sin(e4)*sin(e6) + de1*m6*y6^2*cos(e4)*cos(e6)*sin(e2)*sin(e3)*sin(e4)*sin(e6) + de1*m6*x6^2*cos(e2)*cos(e3)*cos(e4)*cos(e5)^2*cos(e6)*sin(e4)*sin(e6) - 1.0*de1*m6*y6^2*cos(e2)*cos(e3)*cos(e4)*cos(e5)^2*cos(e6)*sin(e4)*sin(e6) - 2.0*de1*m6*x6*y6*cos(e2)*cos(e4)*cos(e6)*sin(e3)*sin(e5)*sin(e6) - 2.0*de1*m6*x6*y6*cos(e3)*cos(e4)*cos(e6)*sin(e2)*sin(e5)*sin(e6) - 1.0*de1*m6*x6^2*cos(e4)*cos(e5)^2*cos(e6)*sin(e2)*sin(e3)*sin(e4)*sin(e6) + de1*m6*y6^2*cos(e4)*cos(e5)^2*cos(e6)*sin(e2)*sin(e3)*sin(e4)*sin(e6) + 4.0*de1*m6*x6*y6*cos(e2)*cos(e3)*cos(e4)^2*cos(e5)*cos(e6)*sin(e6) - 2.0*de1*m6*x6*y6*cos(e2)*cos(e5)*cos(e6)^2*sin(e3)*sin(e4)*sin(e5) - 2.0*de1*m6*x6*y6*cos(e3)*cos(e5)*cos(e6)^2*sin(e2)*sin(e4)*sin(e5) - 4.0*de1*m6*x6*y6*cos(e4)^2*cos(e5)*cos(e6)*sin(e2)*sin(e3)*sin(e6) + 2.0*de1*m6*x6*y6*cos(e2)*cos(e3)*cos(e4)*cos(e5)^2*cos(e6)^2*sin(e4) - 1.0*de1*m6*x6^2*cos(e2)*cos(e5)*cos(e6)*sin(e3)*sin(e4)*sin(e5)*sin(e6) - 1.0*de1*m6*x6^2*cos(e3)*cos(e5)*cos(e6)*sin(e2)*sin(e4)*sin(e5)*sin(e6) - 2.0*de1*m6*x6*y6*cos(e4)*cos(e5)^2*cos(e6)^2*sin(e2)*sin(e3)*sin(e4) + de1*m6*y6^2*cos(e2)*cos(e5)*cos(e6)*sin(e3)*sin(e4)*sin(e5)*sin(e6) + de1*m6*y6^2*cos(e3)*cos(e5)*cos(e6)*sin(e2)*sin(e4)*sin(e5)*sin(e6) - 1.0*de1*m6*y6*z6*cos(e2)*cos(e3)*cos(e4)*cos(e5)*cos(e6)*sin(e4)*sin(e5) - 1.0*de1*m6*x6*z6*cos(e2)*cos(e3)*cos(e4)*cos(e5)*sin(e4)*sin(e5)*sin(e6) + de1*m6*y6*z6*cos(e4)*cos(e5)*cos(e6)*sin(e2)*sin(e3)*sin(e4)*sin(e5) + de1*m6*x6*z6*cos(e4)*cos(e5)*sin(e2)*sin(e3)*sin(e4)*sin(e5)*sin(e6);
C64 = 0.25*I6xx*de4*sin(2.0*e6) - 0.25*I6yy*de4*sin(2.0*e6) - 0.5*I6xx*de5*sin(e5) + 0.5*I6yy*de5*sin(e5) - 1.0*I6zz*de5*sin(e5) + I6xx*de5*cos(e6)^2*sin(e5) - 1.0*I6yy*de5*cos(e6)^2*sin(e5) - 0.25*de4*m6*x6^2*sin(2.0*e6) + 0.25*de4*m6*y6^2*sin(2.0*e6) - 0.5*I6xx*de2*cos(e4)*sin(e5) - 0.5*I6xx*de3*cos(e4)*sin(e5) + 0.5*I6yy*de2*cos(e4)*sin(e5) + 0.5*I6yy*de3*cos(e4)*sin(e5) - 0.5*de5*m6*x6^2*sin(e5) - 1.5*de5*m6*y6^2*sin(e5) - 1.0*de5*m6*x6^2*cos(e6)^2*sin(e5) + de5*m6*y6^2*cos(e6)^2*sin(e5) - 0.5*I6xx*de4*cos(2.0*e5)*cos(e6)*sin(e6) + 0.5*I6yy*de4*cos(2.0*e5)*cos(e6)*sin(e6) - 0.5*de4*m6*x6*y6*cos(2.0*e5) - 0.5*de4*m6*x6*y6*cos(2.0*e6) + 0.5*de2*m6*x6^2*cos(e4)*sin(e5) + 0.5*de3*m6*x6^2*cos(e4)*sin(e5) - 0.5*de2*m6*y6^2*cos(e4)*sin(e5) - 0.5*de3*m6*y6^2*cos(e4)*sin(e5) + I6xx*de2*cos(e4)*cos(e6)^2*sin(e5) + I6xx*de3*cos(e4)*cos(e6)^2*sin(e5) - 1.0*I6yy*de2*cos(e4)*cos(e6)^2*sin(e5) - 1.0*I6yy*de3*cos(e4)*cos(e6)^2*sin(e5) + 0.5*de4*m6*x6^2*cos(2.0*e5)*cos(e6)*sin(e6) - 0.5*de4*m6*y6^2*cos(2.0*e5)*cos(e6)*sin(e6) - 0.5*I6xx*de1*cos(e2)*cos(e3)*sin(e4)*sin(e5) - 1.0*I6xx*de1*cos(e2)*cos(e6)*sin(e3)*sin(e6) - 1.0*I6xx*de1*cos(e3)*cos(e6)*sin(e2)*sin(e6) + 0.5*I6yy*de1*cos(e2)*cos(e3)*sin(e4)*sin(e5) + I6yy*de1*cos(e2)*cos(e6)*sin(e3)*sin(e6) + I6yy*de1*cos(e3)*cos(e6)*sin(e2)*sin(e6) - 0.5*de4*m6*y6*z6*sin(2.0*e5)*cos(e6) + 0.5*I6xx*de1*sin(e2)*sin(e3)*sin(e4)*sin(e5) - 0.5*I6yy*de1*sin(e2)*sin(e3)*sin(e4)*sin(e5) - 0.5*de4*m6*x6*z6*sin(2.0*e5)*sin(e6) - 0.5*d4*de2*m6*x6*cos(e4)*cos(e6) - 0.5*d4*de3*m6*x6*cos(e4)*cos(e6) - 0.5*a1*de1*m6*x6*cos(e6)*sin(e4) + 0.5*d4*de2*m6*y6*cos(e4)*sin(e6) + 0.5*d4*de3*m6*y6*cos(e4)*sin(e6) + de4*m6*x6*y6*cos(2.0*e5)*cos(e6)^2 - 1.5*de5*m6*x6*z6*cos(e5)*cos(e6) + 0.5*a1*de1*m6*y6*sin(e4)*sin(e6) - 1.0*de1*m6*x6*y6*cos(e2)*sin(e3) - 1.0*de1*m6*x6*y6*cos(e3)*sin(e2) - 0.5*de2*m6*y6*z6*cos(e6)*sin(e4) - 0.5*de3*m6*y6*z6*cos(e6)*sin(e4) + 1.5*de5*m6*y6*z6*cos(e5)*sin(e6) + 0.5*de6*m6*y6*z6*cos(e6)*sin(e5) - 1.0*de2*m6*x6^2*cos(e4)*cos(e6)^2*sin(e5) - 1.0*de3*m6*x6^2*cos(e4)*cos(e6)^2*sin(e5) + de2*m6*y6^2*cos(e4)*cos(e6)^2*sin(e5) + de3*m6*y6^2*cos(e4)*cos(e6)^2*sin(e5) - 0.5*de2*m6*x6*z6*sin(e4)*sin(e6) - 0.5*de3*m6*x6*z6*sin(e4)*sin(e6) + 0.5*de6*m6*x6*z6*sin(e5)*sin(e6) - 1.0*I6xx*de2*cos(e5)*cos(e6)*sin(e4)*sin(e5)*sin(e6) - 1.0*I6xx*de3*cos(e5)*cos(e6)*sin(e4)*sin(e5)*sin(e6) + I6yy*de2*cos(e5)*cos(e6)*sin(e4)*sin(e5)*sin(e6) + I6yy*de3*cos(e5)*cos(e6)*sin(e4)*sin(e5)*sin(e6) + 0.5*de1*m6*x6^2*cos(e2)*cos(e3)*sin(e4)*sin(e5) + de1*m6*x6^2*cos(e2)*cos(e6)*sin(e3)*sin(e6) + de1*m6*x6^2*cos(e3)*cos(e6)*sin(e2)*sin(e6) - 0.5*de1*m6*y6^2*cos(e2)*cos(e3)*sin(e4)*sin(e5) - 1.0*de1*m6*y6^2*cos(e2)*cos(e6)*sin(e3)*sin(e6) - 1.0*de1*m6*y6^2*cos(e3)*cos(e6)*sin(e2)*sin(e6) - 0.5*a1*de1*m6*y6*cos(e4)*cos(e5)*cos(e6) - 0.5*de1*m6*x6^2*sin(e2)*sin(e3)*sin(e4)*sin(e5) + 0.5*de1*m6*y6^2*sin(e2)*sin(e3)*sin(e4)*sin(e5) - 0.5*a1*de1*m6*x6*cos(e4)*cos(e5)*sin(e6) + 0.5*a2*de2*m6*x6*cos(e4)*cos(e6)*sin(e3) + I6xx*de1*cos(e2)*cos(e3)*cos(e6)^2*sin(e4)*sin(e5) + I6xx*de1*cos(e2)*cos(e5)^2*cos(e6)*sin(e3)*sin(e6) + I6xx*de1*cos(e3)*cos(e5)^2*cos(e6)*sin(e2)*sin(e6) - 1.0*I6yy*de1*cos(e2)*cos(e3)*cos(e6)^2*sin(e4)*sin(e5) - 1.0*I6yy*de1*cos(e2)*cos(e5)^2*cos(e6)*sin(e3)*sin(e6) - 1.0*I6yy*de1*cos(e3)*cos(e5)^2*cos(e6)*sin(e2)*sin(e6) + 0.5*d4*de2*m6*y6*cos(e5)*cos(e6)*sin(e4) + 0.5*d4*de3*m6*y6*cos(e5)*cos(e6)*sin(e4) - 0.5*de2*m6*x6*z6*cos(e4)*cos(e5)*cos(e6) - 0.5*de3*m6*x6*z6*cos(e4)*cos(e5)*cos(e6) - 0.5*a2*de1*m6*x6*cos(e6)*sin(e2)*sin(e4) - 0.5*a2*de2*m6*y6*cos(e4)*sin(e3)*sin(e6) + 0.5*d4*de2*m6*x6*cos(e5)*sin(e4)*sin(e6) + 0.5*d4*de3*m6*x6*cos(e5)*sin(e4)*sin(e6) + 0.5*de2*m6*y6*z6*cos(e4)*cos(e5)*sin(e6) + 0.5*de3*m6*y6*z6*cos(e4)*cos(e5)*sin(e6) + 0.5*a2*de1*m6*y6*sin(e2)*sin(e4)*sin(e6) - 1.0*I6xx*de1*cos(e6)^2*sin(e2)*sin(e3)*sin(e4)*sin(e5) + I6yy*de1*cos(e6)^2*sin(e2)*sin(e3)*sin(e4)*sin(e5) - 1.0*de2*m6*x6*y6*cos(e5)*sin(e4)*sin(e5) - 1.0*de3*m6*x6*y6*cos(e5)*sin(e4)*sin(e5) + 2.0*de5*m6*x6*y6*cos(e6)*sin(e5)*sin(e6) + de1*m6*x6*y6*cos(e2)*cos(e5)^2*sin(e3) + de1*m6*x6*y6*cos(e3)*cos(e5)^2*sin(e2) + 2.0*de1*m6*x6*y6*cos(e2)*cos(e6)^2*sin(e3) + 2.0*de1*m6*x6*y6*cos(e3)*cos(e6)^2*sin(e2) + de2*m6*y6*z6*cos(e5)^2*cos(e6)*sin(e4) + de3*m6*y6*z6*cos(e5)^2*cos(e6)*sin(e4) + de2*m6*x6*z6*cos(e5)^2*sin(e4)*sin(e6) + de3*m6*x6*z6*cos(e5)^2*sin(e4)*sin(e6) - 2.0*de1*m6*x6*y6*cos(e2)*cos(e5)^2*cos(e6)^2*sin(e3) - 2.0*de1*m6*x6*y6*cos(e3)*cos(e5)^2*cos(e6)^2*sin(e2) + de2*m6*x6^2*cos(e5)*cos(e6)*sin(e4)*sin(e5)*sin(e6) + de3*m6*x6^2*cos(e5)*cos(e6)*sin(e4)*sin(e5)*sin(e6) - 1.0*de2*m6*y6^2*cos(e5)*cos(e6)*sin(e4)*sin(e5)*sin(e6) - 1.0*de3*m6*y6^2*cos(e5)*cos(e6)*sin(e4)*sin(e5)*sin(e6) - 0.5*a2*de1*m6*y6*cos(e4)*cos(e5)*cos(e6)*sin(e2) - 0.5*d4*de1*m6*x6*cos(e2)*cos(e3)*cos(e6)*sin(e4) + 0.5*de1*m6*y6*z6*cos(e2)*cos(e3)*cos(e4)*cos(e6) - 0.5*a3*de1*m6*x6*cos(e2)*cos(e6)*sin(e3)*sin(e4) - 0.5*a3*de1*m6*x6*cos(e3)*cos(e6)*sin(e2)*sin(e4) - 0.5*a2*de1*m6*x6*cos(e4)*cos(e5)*sin(e2)*sin(e6) - 0.5*a2*de2*m6*y6*cos(e5)*cos(e6)*sin(e3)*sin(e4) + 0.5*d4*de1*m6*y6*cos(e2)*cos(e3)*sin(e4)*sin(e6) + 0.5*de1*m6*x6*z6*cos(e2)*cos(e3)*cos(e4)*sin(e6) - 0.5*a2*de2*m6*x6*cos(e5)*sin(e3)*sin(e4)*sin(e6) + 0.5*a3*de1*m6*y6*cos(e2)*sin(e3)*sin(e4)*sin(e6) + 0.5*a3*de1*m6*y6*cos(e3)*sin(e2)*sin(e4)*sin(e6) + 0.5*d4*de1*m6*x6*cos(e6)*sin(e2)*sin(e3)*sin(e4) + 2.0*de2*m6*x6*y6*cos(e4)*cos(e6)*sin(e5)*sin(e6) + 2.0*de3*m6*x6*y6*cos(e4)*cos(e6)*sin(e5)*sin(e6) - 0.5*de1*m6*y6*z6*cos(e4)*cos(e6)*sin(e2)*sin(e3) - 0.5*d4*de1*m6*y6*sin(e2)*sin(e3)*sin(e4)*sin(e6) - 1.0*de1*m6*x6^2*cos(e2)*cos(e3)*cos(e6)^2*sin(e4)*sin(e5) - 1.0*de1*m6*x6^2*cos(e2)*cos(e5)^2*cos(e6)*sin(e3)*sin(e6) - 1.0*de1*m6*x6^2*cos(e3)*cos(e5)^2*cos(e6)*sin(e2)*sin(e6) + de1*m6*y6^2*cos(e2)*cos(e3)*cos(e6)^2*sin(e4)*sin(e5) + de1*m6*y6^2*cos(e2)*cos(e5)^2*cos(e6)*sin(e3)*sin(e6) + de1*m6*y6^2*cos(e3)*cos(e5)^2*cos(e6)*sin(e2)*sin(e6) - 0.5*de1*m6*x6*z6*cos(e4)*sin(e2)*sin(e3)*sin(e6) + de1*m6*x6^2*cos(e6)^2*sin(e2)*sin(e3)*sin(e4)*sin(e5) - 1.0*de1*m6*y6^2*cos(e6)^2*sin(e2)*sin(e3)*sin(e4)*sin(e5) + 2.0*de2*m6*x6*y6*cos(e5)*cos(e6)^2*sin(e4)*sin(e5) + 2.0*de3*m6*x6*y6*cos(e5)*cos(e6)^2*sin(e4)*sin(e5) - 0.5*a3*de1*m6*y6*cos(e2)*cos(e4)*cos(e5)*cos(e6)*sin(e3) - 0.5*a3*de1*m6*y6*cos(e3)*cos(e4)*cos(e5)*cos(e6)*sin(e2) - 0.5*d4*de1*m6*x6*cos(e2)*cos(e3)*cos(e4)*cos(e5)*sin(e6) - 0.5*a3*de1*m6*x6*cos(e2)*cos(e4)*cos(e5)*sin(e3)*sin(e6) - 0.5*a3*de1*m6*x6*cos(e3)*cos(e4)*cos(e5)*sin(e2)*sin(e6) + 0.5*d4*de1*m6*y6*cos(e4)*cos(e5)*cos(e6)*sin(e2)*sin(e3) + de1*m6*x6*y6*cos(e2)*cos(e3)*cos(e4)*cos(e5)*sin(e5) - 0.5*de1*m6*x6*z6*cos(e2)*cos(e3)*cos(e5)*cos(e6)*sin(e4) + 0.5*d4*de1*m6*x6*cos(e4)*cos(e5)*sin(e2)*sin(e3)*sin(e6) + 0.5*de1*m6*y6*z6*cos(e2)*cos(e3)*cos(e5)*sin(e4)*sin(e6) + de1*m6*y6*z6*cos(e2)*cos(e5)*cos(e6)*sin(e3)*sin(e5) + de1*m6*y6*z6*cos(e3)*cos(e5)*cos(e6)*sin(e2)*sin(e5) - 1.0*de1*m6*x6*y6*cos(e4)*cos(e5)*sin(e2)*sin(e3)*sin(e5) + 0.5*de1*m6*x6*z6*cos(e5)*cos(e6)*sin(e2)*sin(e3)*sin(e4) + de1*m6*x6*z6*cos(e2)*cos(e5)*sin(e3)*sin(e5)*sin(e6) + de1*m6*x6*z6*cos(e3)*cos(e5)*sin(e2)*sin(e5)*sin(e6) - 0.5*de1*m6*y6*z6*cos(e5)*sin(e2)*sin(e3)*sin(e4)*sin(e6) - 1.0*de1*m6*y6*z6*cos(e2)*cos(e3)*cos(e4)*cos(e5)^2*cos(e6) - 1.0*de1*m6*x6*z6*cos(e2)*cos(e3)*cos(e4)*cos(e5)^2*sin(e6) + de1*m6*y6*z6*cos(e4)*cos(e5)^2*cos(e6)*sin(e2)*sin(e3) + de1*m6*x6*z6*cos(e4)*cos(e5)^2*sin(e2)*sin(e3)*sin(e6) + I6xx*de1*cos(e2)*cos(e3)*cos(e4)*cos(e5)*cos(e6)*sin(e5)*sin(e6) - 1.0*I6yy*de1*cos(e2)*cos(e3)*cos(e4)*cos(e5)*cos(e6)*sin(e5)*sin(e6) - 1.0*I6xx*de1*cos(e4)*cos(e5)*cos(e6)*sin(e2)*sin(e3)*sin(e5)*sin(e6) + I6yy*de1*cos(e4)*cos(e5)*cos(e6)*sin(e2)*sin(e3)*sin(e5)*sin(e6) - 0.5*d4*de1*m6*y6*cos(e2)*cos(e3)*cos(e4)*cos(e5)*cos(e6) + 2.0*de1*m6*x6*y6*cos(e2)*cos(e3)*cos(e6)*sin(e4)*sin(e5)*sin(e6) - 2.0*de1*m6*x6*y6*cos(e6)*sin(e2)*sin(e3)*sin(e4)*sin(e5)*sin(e6) - 2.0*de1*m6*x6*y6*cos(e2)*cos(e3)*cos(e4)*cos(e5)*cos(e6)^2*sin(e5) + 2.0*de1*m6*x6*y6*cos(e4)*cos(e5)*cos(e6)^2*sin(e2)*sin(e3)*sin(e5) - 1.0*de1*m6*x6^2*cos(e2)*cos(e3)*cos(e4)*cos(e5)*cos(e6)*sin(e5)*sin(e6) + de1*m6*y6^2*cos(e2)*cos(e3)*cos(e4)*cos(e5)*cos(e6)*sin(e5)*sin(e6) + de1*m6*x6^2*cos(e4)*cos(e5)*cos(e6)*sin(e2)*sin(e3)*sin(e5)*sin(e6) - 1.0*de1*m6*y6^2*cos(e4)*cos(e5)*cos(e6)*sin(e2)*sin(e3)*sin(e5)*sin(e6);
C65 = 0.5*I6yy*de5*sin(2.0*e6) - 0.5*I6xx*de5*sin(2.0*e6) - 0.5*I6xx*de4*sin(e5) + 0.5*I6yy*de4*sin(e5) + I6xx*de4*cos(e6)^2*sin(e5) - 1.0*I6yy*de4*cos(e6)^2*sin(e5) + 0.5*de5*m6*x6^2*sin(2.0*e6) - 0.5*de5*m6*y6^2*sin(2.0*e6) + 0.5*I6xx*de2*cos(e5)*sin(e4) + 0.5*I6xx*de3*cos(e5)*sin(e4) - 0.5*I6yy*de2*cos(e5)*sin(e4) - 0.5*I6yy*de3*cos(e5)*sin(e4) + 0.5*de4*m6*x6^2*sin(e5) - 0.5*de4*m6*y6^2*sin(e5) - 1.0*de4*m6*x6^2*cos(e6)^2*sin(e5) + de4*m6*y6^2*cos(e6)^2*sin(e5) - 1.0*I6xx*de2*cos(e4)*cos(e6)*sin(e6) - 1.0*I6xx*de3*cos(e4)*cos(e6)*sin(e6) + I6yy*de2*cos(e4)*cos(e6)*sin(e6) + I6yy*de3*cos(e4)*cos(e6)*sin(e6) + 0.5*I6xx*de1*cos(e2)*sin(e3)*sin(e5) + 0.5*I6xx*de1*cos(e3)*sin(e2)*sin(e5) - 0.5*I6yy*de1*cos(e2)*sin(e3)*sin(e5) - 0.5*I6yy*de1*cos(e3)*sin(e2)*sin(e5) + de5*m6*x6*y6*cos(2.0*e6) - 0.5*de2*m6*x6^2*cos(e5)*sin(e4) - 0.5*de3*m6*x6^2*cos(e5)*sin(e4) + 0.5*de2*m6*y6^2*cos(e5)*sin(e4) + 0.5*de3*m6*y6^2*cos(e5)*sin(e4) - 1.0*I6xx*de2*cos(e5)*cos(e6)^2*sin(e4) - 1.0*I6xx*de3*cos(e5)*cos(e6)^2*sin(e4) + I6yy*de2*cos(e5)*cos(e6)^2*sin(e4) + I6yy*de3*cos(e5)*cos(e6)^2*sin(e4) - 1.0*de2*m6*x6*y6*cos(e4) - 1.0*de3*m6*x6*y6*cos(e4) + 0.5*de6*m6*x6*z6*cos(e6) - 0.5*de6*m6*y6*z6*sin(e6) + 2.0*de2*m6*x6*y6*cos(e4)*cos(e6)^2 + 2.0*de3*m6*x6*y6*cos(e4)*cos(e6)^2 - 0.5*I6xx*de1*cos(e2)*cos(e3)*cos(e4)*cos(e5) + 0.5*I6yy*de1*cos(e2)*cos(e3)*cos(e4)*cos(e5) + 0.5*I6xx*de1*cos(e4)*cos(e5)*sin(e2)*sin(e3) - 0.5*I6yy*de1*cos(e4)*cos(e5)*sin(e2)*sin(e3) + de2*m6*x6^2*cos(e4)*cos(e6)*sin(e6) + de3*m6*x6^2*cos(e4)*cos(e6)*sin(e6) - 1.0*de2*m6*y6^2*cos(e4)*cos(e6)*sin(e6) - 1.0*de3*m6*y6^2*cos(e4)*cos(e6)*sin(e6) - 0.5*de1*m6*x6^2*cos(e2)*sin(e3)*sin(e5) - 0.5*de1*m6*x6^2*cos(e3)*sin(e2)*sin(e5) + 0.5*de1*m6*y6^2*cos(e2)*sin(e3)*sin(e5) + 0.5*de1*m6*y6^2*cos(e3)*sin(e2)*sin(e5) + 0.5*a3*de2*m6*y6*cos(e5)*cos(e6) + 0.5*a3*de3*m6*y6*cos(e5)*cos(e6) + 0.5*a3*de2*m6*x6*cos(e5)*sin(e6) + 0.5*a3*de3*m6*x6*cos(e5)*sin(e6) - 1.0*I6xx*de1*cos(e2)*cos(e6)^2*sin(e3)*sin(e5) - 1.0*I6xx*de1*cos(e3)*cos(e6)^2*sin(e2)*sin(e5) + I6yy*de1*cos(e2)*cos(e6)^2*sin(e3)*sin(e5) + I6yy*de1*cos(e3)*cos(e6)^2*sin(e2)*sin(e5) - 0.5*de4*m6*x6*z6*cos(e5)*cos(e6) + 0.5*de4*m6*y6*z6*cos(e5)*sin(e6) + de2*m6*x6^2*cos(e5)*cos(e6)^2*sin(e4) + de3*m6*x6^2*cos(e5)*cos(e6)^2*sin(e4) - 1.0*de2*m6*y6^2*cos(e5)*cos(e6)^2*sin(e4) - 1.0*de3*m6*y6^2*cos(e5)*cos(e6)^2*sin(e4) - 1.0*I6xx*de1*cos(e2)*cos(e3)*cos(e6)*sin(e4)*sin(e6) + I6yy*de1*cos(e2)*cos(e3)*cos(e6)*sin(e4)*sin(e6) + 0.5*de1*m6*x6^2*cos(e2)*cos(e3)*cos(e4)*cos(e5) - 0.5*de1*m6*y6^2*cos(e2)*cos(e3)*cos(e4)*cos(e5) + I6xx*de1*cos(e6)*sin(e2)*sin(e3)*sin(e4)*sin(e6) - 1.0*I6yy*de1*cos(e6)*sin(e2)*sin(e3)*sin(e4)*sin(e6) - 0.5*de1*m6*x6^2*cos(e4)*cos(e5)*sin(e2)*sin(e3) + 0.5*de1*m6*y6^2*cos(e4)*cos(e5)*sin(e2)*sin(e3) + I6xx*de1*cos(e2)*cos(e3)*cos(e4)*cos(e5)*cos(e6)^2 - 1.0*I6yy*de1*cos(e2)*cos(e3)*cos(e4)*cos(e5)*cos(e6)^2 + 0.5*a2*de2*m6*y6*cos(e3)*cos(e5)*cos(e6) + 0.5*a2*de2*m6*x6*cos(e3)*cos(e5)*sin(e6) - 1.0*I6xx*de1*cos(e4)*cos(e5)*cos(e6)^2*sin(e2)*sin(e3) + I6yy*de1*cos(e4)*cos(e5)*cos(e6)^2*sin(e2)*sin(e3) + 0.5*d4*de2*m6*y6*cos(e4)*cos(e6)*sin(e5) + 0.5*d4*de3*m6*y6*cos(e4)*cos(e6)*sin(e5) + 0.5*a1*de1*m6*y6*cos(e6)*sin(e4)*sin(e5) + 0.5*d4*de2*m6*x6*cos(e4)*sin(e5)*sin(e6) + 0.5*d4*de3*m6*x6*cos(e4)*sin(e5)*sin(e6) - 1.0*de1*m6*x6*y6*cos(e2)*cos(e3)*sin(e4) + 0.5*a1*de1*m6*x6*sin(e4)*sin(e5)*sin(e6) + 2.0*de4*m6*x6*y6*cos(e6)*sin(e5)*sin(e6) - 0.5*de2*m6*x6*z6*cos(e6)*sin(e4)*sin(e5) - 0.5*de3*m6*x6*z6*cos(e6)*sin(e4)*sin(e5) + de1*m6*x6^2*cos(e2)*cos(e6)^2*sin(e3)*sin(e5) + de1*m6*x6^2*cos(e3)*cos(e6)^2*sin(e2)*sin(e5) - 1.0*de1*m6*y6^2*cos(e2)*cos(e6)^2*sin(e3)*sin(e5) - 1.0*de1*m6*y6^2*cos(e3)*cos(e6)^2*sin(e2)*sin(e5) + de1*m6*x6*y6*sin(e2)*sin(e3)*sin(e4) + 0.5*de2*m6*y6*z6*sin(e4)*sin(e5)*sin(e6) + 0.5*de3*m6*y6*z6*sin(e4)*sin(e5)*sin(e6) + de1*m6*x6^2*cos(e2)*cos(e3)*cos(e6)*sin(e4)*sin(e6) - 1.0*de1*m6*y6^2*cos(e2)*cos(e3)*cos(e6)*sin(e4)*sin(e6) - 1.0*de1*m6*x6^2*cos(e6)*sin(e2)*sin(e3)*sin(e4)*sin(e6) + de1*m6*y6^2*cos(e6)*sin(e2)*sin(e3)*sin(e4)*sin(e6) - 0.5*a2*de2*m6*y6*cos(e4)*cos(e6)*sin(e3)*sin(e5) - 1.0*de1*m6*x6^2*cos(e2)*cos(e3)*cos(e4)*cos(e5)*cos(e6)^2 + de1*m6*y6^2*cos(e2)*cos(e3)*cos(e4)*cos(e5)*cos(e6)^2 + 0.5*de1*m6*x6*z6*cos(e2)*cos(e5)*cos(e6)*sin(e3) + 0.5*de1*m6*x6*z6*cos(e3)*cos(e5)*cos(e6)*sin(e2) - 0.5*a2*de2*m6*x6*cos(e4)*sin(e3)*sin(e5)*sin(e6) + 0.5*a2*de1*m6*y6*cos(e6)*sin(e2)*sin(e4)*sin(e5) - 2.0*de2*m6*x6*y6*cos(e5)*cos(e6)*sin(e4)*sin(e6) - 2.0*de3*m6*x6*y6*cos(e5)*cos(e6)*sin(e4)*sin(e6) - 0.5*de1*m6*y6*z6*cos(e2)*cos(e5)*sin(e3)*sin(e6) - 0.5*de1*m6*y6*z6*cos(e3)*cos(e5)*sin(e2)*sin(e6) + 0.5*a2*de1*m6*x6*sin(e2)*sin(e4)*sin(e5)*sin(e6) + de1*m6*x6^2*cos(e4)*cos(e5)*cos(e6)^2*sin(e2)*sin(e3) - 1.0*de1*m6*y6^2*cos(e4)*cos(e5)*cos(e6)^2*sin(e2)*sin(e3) + 2.0*de1*m6*x6*y6*cos(e2)*cos(e3)*cos(e6)^2*sin(e4) - 2.0*de1*m6*x6*y6*cos(e6)^2*sin(e2)*sin(e3)*sin(e4) + 0.5*d4*de1*m6*y6*cos(e2)*cos(e3)*cos(e6)*sin(e4)*sin(e5) + 0.5*de1*m6*x6*z6*cos(e2)*cos(e3)*cos(e4)*cos(e6)*sin(e5) + 0.5*a3*de1*m6*y6*cos(e2)*cos(e6)*sin(e3)*sin(e4)*sin(e5) + 0.5*a3*de1*m6*y6*cos(e3)*cos(e6)*sin(e2)*sin(e4)*sin(e5) + 0.5*d4*de1*m6*x6*cos(e2)*cos(e3)*sin(e4)*sin(e5)*sin(e6) - 0.5*de1*m6*y6*z6*cos(e2)*cos(e3)*cos(e4)*sin(e5)*sin(e6) + 0.5*a3*de1*m6*x6*cos(e2)*sin(e3)*sin(e4)*sin(e5)*sin(e6) + 0.5*a3*de1*m6*x6*cos(e3)*sin(e2)*sin(e4)*sin(e5)*sin(e6) - 0.5*d4*de1*m6*y6*cos(e6)*sin(e2)*sin(e3)*sin(e4)*sin(e5) - 2.0*de1*m6*x6*y6*cos(e2)*cos(e6)*sin(e3)*sin(e5)*sin(e6) - 2.0*de1*m6*x6*y6*cos(e3)*cos(e6)*sin(e2)*sin(e5)*sin(e6) - 0.5*de1*m6*x6*z6*cos(e4)*cos(e6)*sin(e2)*sin(e3)*sin(e5) - 0.5*d4*de1*m6*x6*sin(e2)*sin(e3)*sin(e4)*sin(e5)*sin(e6) + 0.5*de1*m6*y6*z6*cos(e4)*sin(e2)*sin(e3)*sin(e5)*sin(e6) - 2.0*de1*m6*x6*y6*cos(e4)*cos(e5)*cos(e6)*sin(e2)*sin(e3)*sin(e6) + 2.0*de1*m6*x6*y6*cos(e2)*cos(e3)*cos(e4)*cos(e5)*cos(e6)*sin(e6);
C66 = -(m6*(de5*x6*z6*cos(e6) - 1.0*de5*y6*z6*sin(e6) + a1*de1*y6*cos(e4)*cos(e6) + a1*de1*x6*cos(e4)*sin(e6) - 1.0*a3*de2*x6*cos(e6)*sin(e5) - 1.0*a3*de3*x6*cos(e6)*sin(e5) - 1.0*d4*de2*y6*cos(e6)*sin(e4) - 1.0*d4*de3*y6*cos(e6)*sin(e4) + de2*x6*z6*cos(e4)*cos(e6) + de3*x6*z6*cos(e4)*cos(e6) + a3*de2*y6*sin(e5)*sin(e6) + a3*de3*y6*sin(e5)*sin(e6) - 1.0*d4*de2*x6*sin(e4)*sin(e6) - 1.0*d4*de3*x6*sin(e4)*sin(e6) - 1.0*de2*y6*z6*cos(e4)*sin(e6) - 1.0*de3*y6*z6*cos(e4)*sin(e6) + de4*y6*z6*cos(e6)*sin(e5) + de4*x6*z6*sin(e5)*sin(e6) + a1*de1*x6*cos(e5)*cos(e6)*sin(e4) - 1.0*a2*de2*x6*cos(e3)*cos(e6)*sin(e5) + a2*de1*y6*cos(e4)*cos(e6)*sin(e2) - 1.0*d4*de2*y6*cos(e4)*cos(e5)*sin(e6) - 1.0*d4*de3*y6*cos(e4)*cos(e5)*sin(e6) + a2*de1*x6*cos(e4)*sin(e2)*sin(e6) - 1.0*a1*de1*y6*cos(e5)*sin(e4)*sin(e6) + a2*de2*y6*cos(e6)*sin(e3)*sin(e4) + a2*de2*y6*cos(e3)*sin(e5)*sin(e6) - 1.0*de2*y6*z6*cos(e5)*cos(e6)*sin(e4) - 1.0*de3*y6*z6*cos(e5)*cos(e6)*sin(e4) + a2*de2*x6*sin(e3)*sin(e4)*sin(e6) - 1.0*de2*x6*z6*cos(e5)*sin(e4)*sin(e6) - 1.0*de3*x6*z6*cos(e5)*sin(e4)*sin(e6) + d4*de2*x6*cos(e4)*cos(e5)*cos(e6) + d4*de3*x6*cos(e4)*cos(e5)*cos(e6) - 1.0*de1*x6*z6*cos(e6)*sin(e2)*sin(e3)*sin(e4) - 1.0*de1*x6*z6*cos(e2)*sin(e3)*sin(e5)*sin(e6) - 1.0*de1*x6*z6*cos(e3)*sin(e2)*sin(e5)*sin(e6) + de1*y6*z6*sin(e2)*sin(e3)*sin(e4)*sin(e6) + d4*de1*y6*cos(e2)*cos(e3)*cos(e4)*cos(e6) - 1.0*a2*de2*x6*cos(e4)*cos(e5)*cos(e6)*sin(e3) + a3*de1*y6*cos(e2)*cos(e4)*cos(e6)*sin(e3) + a3*de1*y6*cos(e3)*cos(e4)*cos(e6)*sin(e2) + d4*de1*x6*cos(e2)*cos(e3)*cos(e4)*sin(e6) + a3*de1*x6*cos(e2)*cos(e4)*sin(e3)*sin(e6) + a3*de1*x6*cos(e3)*cos(e4)*sin(e2)*sin(e6) + a2*de1*x6*cos(e5)*cos(e6)*sin(e2)*sin(e4) + a2*de2*y6*cos(e4)*cos(e5)*sin(e3)*sin(e6) - 1.0*d4*de1*y6*cos(e4)*cos(e6)*sin(e2)*sin(e3) + de1*x6*z6*cos(e2)*cos(e3)*cos(e6)*sin(e4) - 1.0*a2*de1*y6*cos(e5)*sin(e2)*sin(e4)*sin(e6) - 1.0*d4*de1*x6*cos(e4)*sin(e2)*sin(e3)*sin(e6) - 1.0*de1*y6*z6*cos(e2)*cos(e3)*sin(e4)*sin(e6) - 1.0*de1*y6*z6*cos(e2)*cos(e6)*sin(e3)*sin(e5) - 1.0*de1*y6*z6*cos(e3)*cos(e6)*sin(e2)*sin(e5) + d4*de1*x6*cos(e2)*cos(e3)*cos(e5)*cos(e6)*sin(e4) + de1*y6*z6*cos(e2)*cos(e3)*cos(e4)*cos(e5)*cos(e6) + a3*de1*x6*cos(e2)*cos(e5)*cos(e6)*sin(e3)*sin(e4) + a3*de1*x6*cos(e3)*cos(e5)*cos(e6)*sin(e2)*sin(e4) - 1.0*d4*de1*y6*cos(e2)*cos(e3)*cos(e5)*sin(e4)*sin(e6) + de1*x6*z6*cos(e2)*cos(e3)*cos(e4)*cos(e5)*sin(e6) - 1.0*a3*de1*y6*cos(e2)*cos(e5)*sin(e3)*sin(e4)*sin(e6) - 1.0*a3*de1*y6*cos(e3)*cos(e5)*sin(e2)*sin(e4)*sin(e6) - 1.0*d4*de1*x6*cos(e5)*cos(e6)*sin(e2)*sin(e3)*sin(e4) - 1.0*de1*y6*z6*cos(e4)*cos(e5)*cos(e6)*sin(e2)*sin(e3) + d4*de1*y6*cos(e5)*sin(e2)*sin(e3)*sin(e4)*sin(e6) - 1.0*de1*x6*z6*cos(e4)*cos(e5)*sin(e2)*sin(e3)*sin(e6)))/2;

C = [C11,C121+C122+C123,C131+C132+C133,C141+C142,C15,C16;
	 C211+C212+C213+C214+C215+C216,C22,C23,C24,C25,C26;
	 C311+C312+C313+C314+C315,C32,C33,C34,C35,C36;
	 C411+C412+C413+C414,C421+C422,C431+C432,C44,C45,C46;
	 C511+C512+C513+C514,C52,C53,C54,C55,C56;
	 C611+C612,C62,C63,C64,C65,C66;];

G = ...
[0;
(g*(2*a2*m3*sin(e2) + 2*a2*m4*sin(e2) + 2*a2*m5*sin(e2) + 2*a2*m6*sin(e2) + 2*m2*y2*cos(e2) + 2*m2*x2*sin(e2) + 2*d4*m4*cos(e2 + e3) + 2*d4*m5*cos(e2 + e3) + 2*d4*m6*cos(e2 + e3) + 2*a3*m4*sin(e2 + e3) + 2*a3*m5*sin(e2 + e3) + 2*a3*m6*sin(e2 + e3) + 2*m3*y3*cos(e2 + e3) + 2*m4*z4*cos(e2 + e3) + 2*m3*x3*sin(e2 + e3) + m5*x5*cos(e4 + e5)*sin(e2 + e3) + m6*x6*cos(e4 + e6)*sin(e2 + e3) - m5*y5*sin(e2 + e3)*sin(e4 + e5) - m6*y6*sin(e2 + e3)*sin(e4 + e6) - m6*z6*sin(e2 + e3)*sin(e4 + e5) + 2*m5*y5*cos(e2 + e3)*cos(e5) + 2*m6*z6*cos(e2 + e3)*cos(e5) + 2*m4*x4*sin(e2 + e3)*cos(e4) + 2*m5*x5*cos(e2 + e3)*sin(e5) - 2*m4*y4*sin(e2 + e3)*sin(e4) + 2*m5*z5*sin(e2 + e3)*sin(e4) + m5*x5*sin(e2 + e3)*cos(e4 - e5) - m6*x6*sin(e2 + e3)*cos(e4 - e6) + m5*y5*sin(e2 + e3)*sin(e4 - e5) - m6*y6*sin(e2 + e3)*sin(e4 - e6) + m6*z6*sin(e2 + e3)*sin(e4 - e5) + m6*x6*cos(e4 + e5)*sin(e2 + e3)*cos(e6) - m6*y6*cos(e4 + e5)*sin(e2 + e3)*sin(e6) + 2*m6*x6*cos(e2 + e3)*cos(e6)*sin(e5) - 2*m6*y6*cos(e2 + e3)*sin(e5)*sin(e6) + m6*x6*sin(e2 + e3)*cos(e6)*cos(e4 - e5) - m6*y6*sin(e2 + e3)*sin(e6)*cos(e4 - e5)))/2;
d4*g*m4*cos(e2 + e3) + d4*g*m5*cos(e2 + e3) + d4*g*m6*cos(e2 + e3) + a3*g*m4*sin(e2 + e3) + a3*g*m5*sin(e2 + e3) + a3*g*m6*sin(e2 + e3) + g*m3*y3*cos(e2 + e3) + g*m4*z4*cos(e2 + e3) + g*m3*x3*sin(e2 + e3) + g*m5*y5*cos(e2 + e3)*cos(e5) + g*m6*z6*cos(e2 + e3)*cos(e5) + g*m4*x4*sin(e2 + e3)*cos(e4) + g*m5*x5*cos(e2 + e3)*sin(e5) - g*m4*y4*sin(e2 + e3)*sin(e4) + g*m5*z5*sin(e2 + e3)*sin(e4) + g*m5*x5*sin(e2 + e3)*cos(e4)*cos(e5) + g*m6*x6*cos(e2 + e3)*cos(e6)*sin(e5) - g*m5*y5*sin(e2 + e3)*cos(e4)*sin(e5) - g*m6*y6*sin(e2 + e3)*cos(e6)*sin(e4) - g*m6*y6*cos(e2 + e3)*sin(e5)*sin(e6) - g*m6*z6*sin(e2 + e3)*cos(e4)*sin(e5) - g*m6*x6*sin(e2 + e3)*sin(e4)*sin(e6) + g*m6*x6*sin(e2 + e3)*cos(e4)*cos(e5)*cos(e6) - g*m6*y6*sin(e2 + e3)*cos(e4)*cos(e5)*sin(e6);
g*cos(e2 + e3)*(m4*y4*cos(e4) - m5*z5*cos(e4) + m4*x4*sin(e4) + m6*y6*cos(e4)*cos(e6) + m5*x5*cos(e5)*sin(e4) + m6*x6*cos(e4)*sin(e6) - m5*y5*sin(e4)*sin(e5) - m6*z6*sin(e4)*sin(e5) + m6*x6*cos(e5)*cos(e6)*sin(e4) - m6*y6*cos(e5)*sin(e4)*sin(e6));
g*m5*(x5*sin(e2 + e3)*cos(e5) - y5*sin(e2 + e3)*sin(e5) + x5*cos(e2 + e3)*cos(e4)*sin(e5) + y5*cos(e2 + e3)*cos(e4)*cos(e5)) - g*m6*(z6*(sin(e2 + e3)*sin(e5) - cos(e2 + e3)*cos(e4)*cos(e5)) - x6*cos(e6)*(sin(e2 + e3)*cos(e5) + cos(e2 + e3)*cos(e4)*sin(e5)) + y6*sin(e6)*(sin(e2 + e3)*cos(e5) + cos(e2 + e3)*cos(e4)*sin(e5)));
-g*m6*(y6*(cos(e2 + e3)*sin(e4)*sin(e6) + sin(e2 + e3)*cos(e6)*sin(e5) - cos(e2 + e3)*cos(e4)*cos(e5)*cos(e6)) - x6*(cos(e2 + e3)*cos(e6)*sin(e4) - sin(e2 + e3)*sin(e5)*sin(e6) + cos(e2 + e3)*cos(e4)*cos(e5)*sin(e6)))];


J = ...
[ d4*sin(e1)*sin(e2)*sin(e3) - a2*sin(e1)*sin(e2) - d4*cos(e2)*cos(e3)*sin(e1) - a3*cos(e2)*sin(e1)*sin(e3) - a3*cos(e3)*sin(e1)*sin(e2) - d7*cos(e1)*sin(e4)*sin(e5) - a1*sin(e1) - d7*cos(e2)*cos(e3)*cos(e5)*sin(e1) + d7*cos(e5)*sin(e1)*sin(e2)*sin(e3) + d7*cos(e2)*cos(e4)*sin(e1)*sin(e3)*sin(e5) + d7*cos(e3)*cos(e4)*sin(e1)*sin(e2)*sin(e5), -cos(e1)*(d4*cos(e2)*sin(e3) - a3*cos(e2)*cos(e3) - a2*cos(e2) + d4*cos(e3)*sin(e2) + a3*sin(e2)*sin(e3) + d7*cos(e2)*cos(e5)*sin(e3) + d7*cos(e3)*cos(e5)*sin(e2) + d7*cos(e2)*cos(e3)*cos(e4)*sin(e5) - d7*cos(e4)*sin(e2)*sin(e3)*sin(e5)), -cos(e1)*(d4*cos(e2)*sin(e3) - a3*cos(e2)*cos(e3) + d4*cos(e3)*sin(e2) + a3*sin(e2)*sin(e3) + d7*cos(e2)*cos(e5)*sin(e3) + d7*cos(e3)*cos(e5)*sin(e2) + d7*cos(e2)*cos(e3)*cos(e4)*sin(e5) - d7*cos(e4)*sin(e2)*sin(e3)*sin(e5)), d7*sin(e5)*(cos(e1)*cos(e2)*sin(e3)*sin(e4) - cos(e4)*sin(e1) + cos(e1)*cos(e3)*sin(e2)*sin(e4)), d7*cos(e1)*sin(e2)*sin(e3)*sin(e5) - d7*cos(e1)*cos(e2)*cos(e3)*sin(e5) - d7*cos(e5)*sin(e1)*sin(e4) - d7*cos(e1)*cos(e2)*cos(e4)*cos(e5)*sin(e3) - d7*cos(e1)*cos(e3)*cos(e4)*cos(e5)*sin(e2),                                                                                                                            0;
  a1*cos(e1) + a2*cos(e1)*sin(e2) + d4*cos(e1)*cos(e2)*cos(e3) + a3*cos(e1)*cos(e2)*sin(e3) + a3*cos(e1)*cos(e3)*sin(e2) - d4*cos(e1)*sin(e2)*sin(e3) - d7*sin(e1)*sin(e4)*sin(e5) + d7*cos(e1)*cos(e2)*cos(e3)*cos(e5) - d7*cos(e1)*cos(e5)*sin(e2)*sin(e3) - d7*cos(e1)*cos(e2)*cos(e4)*sin(e3)*sin(e5) - d7*cos(e1)*cos(e3)*cos(e4)*sin(e2)*sin(e5), -sin(e1)*(d4*cos(e2)*sin(e3) - a3*cos(e2)*cos(e3) - a2*cos(e2) + d4*cos(e3)*sin(e2) + a3*sin(e2)*sin(e3) + d7*cos(e2)*cos(e5)*sin(e3) + d7*cos(e3)*cos(e5)*sin(e2) + d7*cos(e2)*cos(e3)*cos(e4)*sin(e5) - d7*cos(e4)*sin(e2)*sin(e3)*sin(e5)), -sin(e1)*(d4*cos(e2)*sin(e3) - a3*cos(e2)*cos(e3) + d4*cos(e3)*sin(e2) + a3*sin(e2)*sin(e3) + d7*cos(e2)*cos(e5)*sin(e3) + d7*cos(e3)*cos(e5)*sin(e2) + d7*cos(e2)*cos(e3)*cos(e4)*sin(e5) - d7*cos(e4)*sin(e2)*sin(e3)*sin(e5)), d7*sin(e5)*(cos(e1)*cos(e4) + cos(e2)*sin(e1)*sin(e3)*sin(e4) + cos(e3)*sin(e1)*sin(e2)*sin(e4)), d7*cos(e1)*cos(e5)*sin(e4) - d7*cos(e2)*cos(e3)*sin(e1)*sin(e5) + d7*sin(e1)*sin(e2)*sin(e3)*sin(e5) - d7*cos(e2)*cos(e4)*cos(e5)*sin(e1)*sin(e3) - d7*cos(e3)*cos(e4)*cos(e5)*sin(e1)*sin(e2),                                                                                                                            0;
                                                                                                                                                                                                                                                                                                                                                     0,            d4*sin(e2)*sin(e3) - d4*cos(e2)*cos(e3) - a3*cos(e2)*sin(e3) - a3*cos(e3)*sin(e2) - a2*sin(e2) - d7*cos(e2)*cos(e3)*cos(e5) + d7*cos(e5)*sin(e2)*sin(e3) + d7*cos(e2)*cos(e4)*sin(e3)*sin(e5) + d7*cos(e3)*cos(e4)*sin(e2)*sin(e5),            d4*sin(e2)*sin(e3) - a3*cos(e2)*sin(e3) - a3*cos(e3)*sin(e2) - d4*cos(e2)*cos(e3) - d7*cos(e2)*cos(e3)*cos(e5) + d7*cos(e5)*sin(e2)*sin(e3) + d7*cos(e2)*cos(e4)*sin(e3)*sin(e5) + d7*cos(e3)*cos(e4)*sin(e2)*sin(e5),                                                                  d7*cos(e2 + e3)*sin(e4)*sin(e5),                                                              d7*cos(e2)*sin(e3)*sin(e5) + d7*cos(e3)*sin(e2)*sin(e5) - d7*cos(e2)*cos(e3)*cos(e4)*cos(e5) + d7*cos(e4)*cos(e5)*sin(e2)*sin(e3),                                                                                                                            0;
                                                                                                                                                                                                                                                                                                                                                     0,                                                                                                                                                                                                                                      -sin(e1),                                                                                                                                                                                                                         -sin(e1),                                                                             cos(e2 + e3)*cos(e1),                                                                                                            cos(e1)*cos(e2)*sin(e3)*sin(e4) - cos(e4)*sin(e1) + cos(e1)*cos(e3)*sin(e2)*sin(e4), cos(e2 + e3)*cos(e1)*cos(e5) - sin(e5)*(sin(e1)*sin(e4) + cos(e1)*cos(e2)*cos(e4)*sin(e3) + cos(e1)*cos(e3)*cos(e4)*sin(e2));
                                                                                                                                                                                                                                                                                                                                                     0,                                                                                                                                                                                                                                       cos(e1),                                                                                                                                                                                                                          cos(e1),                                                                             cos(e2 + e3)*sin(e1),                                                                                                            cos(e1)*cos(e4) + cos(e2)*sin(e1)*sin(e3)*sin(e4) + cos(e3)*sin(e1)*sin(e2)*sin(e4), cos(e2 + e3)*cos(e5)*sin(e1) - sin(e5)*(cos(e2)*cos(e4)*sin(e1)*sin(e3) - cos(e1)*sin(e4) + cos(e3)*cos(e4)*sin(e1)*sin(e2));                                                                                                                                                                                                                                                                                                                                                   1,                                                                                                                                                                                                                                             0,                                                                                                                                                                                                                                0,                                                                                    -sin(e2 + e3),                                                                                                                                                                           cos(e2 + e3)*sin(e4),                                                                        - sin(e2 + e3)*cos(e5) - cos(e2 + e3)*cos(e4)*sin(e5)];
%%
% V = [V1+5*dt1;V2+5*dt2;V3+5*dt3];
de = [de1;de2;de3;de4;de5;de6];
% V = C*de;
% M_inv = inv(M);
% c = 0;
% b = 10;
% Fe = 0*[1;1;1;1;1;1];
F = c*sign(de) + b*de + J'*Fe ;
dde = M\(t-C*de-G-F);
